simulink model "myo_sfun_one_myo_imu_emg"  (R2019a)
(part 6 of 12)

  "IW{2,1}(425,:)'" : Constant  Value=[1.908802925279713402773040797910653054714202880859375;-1.2138358984813477636777179213822819292545318603515625;0.01503844005797187570461215244677077862434089183807373046875;-1.5358594813991690575250004258123226463794708251953125;-0.59196391028480765950092745697475038468837738037109375;1.2715516743513524122732860632822848856449127197265625;1.2233297305976738034161144241807051002979278564453125;-0.5289314826547693026981278308085165917873382568359375]
      mask Display: e = 0.06;c1 = [120 150 230]/255;c2 = ([120 150 230]+0)/383;c3 = ([120 150 230]+128)/383;patch([0 1 1 0],[0 0 1 1],c1);patch([0 1 1 1-e 1-e 0+e],[0 0 1 1-e 0+e 0+e],c2);patch([0 0 1 1-e 0+e 0+e],[0 1 1 1-e 1-e 0+e],c3);plot([0 1 1 0 0],[0 0 1 1 0]);disp('weights');
  "IW{2,1}(426,:)'" : Constant  Value=[1.076656286956270580645877998904325067996978759765625;-0.8088007748125767282232345678494311869144439697265625;0.67060454814467396200683424467570148408412933349609375;0.88562860336622473145240519443177618086338043212890625;-1.9562657272639487615606412873603403568267822265625;-1.9554189585665968653671598076471127569675445556640625;-0.58641998996341160310663553900667466223239898681640625;0.269580957964742629062726564370677806437015533447265625]
      mask Display: e = 0.06;c1 = [120 150 230]/255;c2 = ([120 150 230]+0)/383;c3 = ([120 150 230]+128)/383;patch([0 1 1 0],[0 0 1 1],c1);patch([0 1 1 1-e 1-e 0+e],[0 0 1 1-e 0+e 0+e],c2);patch([0 0 1 1-e 0+e 0+e],[0 1 1 1-e 1-e 0+e],c3);plot([0 1 1 0 0],[0 0 1 1 0]);disp('weights');
  "IW{2,1}(427,:)'" : Constant  Value=[-0.721042740842791740618622498004697263240814208984375;0.79648621538253194795942135897348634898662567138671875;-0.53684047654335553811932868484291248023509979248046875;0.42689430211453827102019431549706496298313140869140625;2.549203011698739640422672891872934997081756591796875;0.3353743207324175745753791488823480904102325439453125;1.3664100055677750322757901813019998371601104736328125;-0.9924099379392383735165594771387986838817596435546875]
      mask Display: e = 0.06;c1 = [120 150 230]/255;c2 = ([120 150 230]+0)/383;c3 = ([120 150 230]+128)/383;patch([0 1 1 0],[0 0 1 1],c1);patch([0 1 1 1-e 1-e 0+e],[0 0 1 1-e 0+e 0+e],c2);patch([0 0 1 1-e 0+e 0+e],[0 1 1 1-e 1-e 0+e],c3);plot([0 1 1 0 0],[0 0 1 1 0]);disp('weights');
  "IW{2,1}(428,:)'" : Constant  Value=[1.2634311689343726836654013823135755956172943115234375;1.499519406449823843985313942539505660533905029296875;-0.8822519927699061792480961230467073619365692138671875;-0.0549891942636861752458088403727742843329906463623046875;-1.5362747666262255297198180414852686226367950439453125;-1.092163209413707480877064881497062742710113525390625;0.5684544617956106549172545783221721649169921875;1.6019203633066683156727094683446921408176422119140625]
      mask Display: e = 0.06;c1 = [120 150 230]/255;c2 = ([120 150 230]+0)/383;c3 = ([120 150 230]+128)/383;patch([0 1 1 0],[0 0 1 1],c1);patch([0 1 1 1-e 1-e 0+e],[0 0 1 1-e 0+e 0+e],c2);patch([0 0 1 1-e 0+e 0+e],[0 1 1 1-e 1-e 0+e],c3);plot([0 1 1 0 0],[0 0 1 1 0]);disp('weights');
  "IW{2,1}(429,:)'" : Constant  Value=[0.08693070549592145368489326529015670530498027801513671875;-1.518156541460599751047766403644345700740814208984375;-1.4111017266934429148506069395807571709156036376953125;2.2271029883890012257552371011115610599517822265625;-0.9991528979578829794405692155123688280582427978515625;0.024328099958265798907763866054665413685142993927001953125;-0.2054258345516097872263117096736095845699310302734375;0.7659566339452936745146871544420719146728515625]
      mask Display: e = 0.06;c1 = [120 150 230]/255;c2 = ([120 150 230]+0)/383;c3 = ([120 150 230]+128)/383;patch([0 1 1 0],[0 0 1 1],c1);patch([0 1 1 1-e 1-e 0+e],[0 0 1 1-e 0+e 0+e],c2);patch([0 0 1 1-e 0+e 0+e],[0 1 1 1-e 1-e 0+e],c3);plot([0 1 1 0 0],[0 0 1 1 0]);disp('weights');
  "IW{2,1}(43,:)'" : Constant  Value=[1.970097053050870794521642892505042254924774169921875;0.61319693162176391876272418812732212245464324951171875;-1.11470914765594297790585187613032758235931396484375;0.2366872070900522817549216370025533251464366912841796875;-1.507392518889222099431890455889515578746795654296875;1.7794743719183812036277458901167847216129302978515625;0.29415914149666377852554433047771453857421875;-0.66480034795872899877622330677695572376251220703125]
      mask Display: e = 0.06;c1 = [120 150 230]/255;c2 = ([120 150 230]+0)/383;c3 = ([120 150 230]+128)/383;patch([0 1 1 0],[0 0 1 1],c1);patch([0 1 1 1-e 1-e 0+e],[0 0 1 1-e 0+e 0+e],c2);patch([0 0 1 1-e 0+e 0+e],[0 1 1 1-e 1-e 0+e],c3);plot([0 1 1 0 0],[0 0 1 1 0]);disp('weights');
  "IW{2,1}(430,:)'" : Constant  Value=[0.91229328205142434793373240609071217477321624755859375;1.8134784160849555245675901460344903171062469482421875;1.8692781171544383678195799802779220044612884521484375;0.035866898596928382947357505372565356083214282989501953125;1.17660347229219208742279079160653054714202880859375;0.1717013531981310403562446253999951295554637908935546875;1.34724376949878621445577664417214691638946533203125;0.43452940443224041811021152170724235475063323974609375]
      mask Display: e = 0.06;c1 = [120 150 230]/255;c2 = ([120 150 230]+0)/383;c3 = ([120 150 230]+128)/383;patch([0 1 1 0],[0 0 1 1],c1);patch([0 1 1 1-e 1-e 0+e],[0 0 1 1-e 0+e 0+e],c2);patch([0 0 1 1-e 0+e 0+e],[0 1 1 1-e 1-e 0+e],c3);plot([0 1 1 0 0],[0 0 1 1 0]);disp('weights');
  "IW{2,1}(431,:)'" : Constant  Value=[1.7686581181827201181278041985933668911457061767578125;-1.601690710654345206620519093121401965618133544921875;-1.4180860902058913808332363259978592395782470703125;-1.18832699803570296381849402678199112415313720703125;0.2237601474155433700641282257493003271520137786865234375;0.65218668674513879945919825331657193601131439208984375;-0.88845803596487160636030466775991953909397125244140625;0.90809653286696201401895223170868121087551116943359375]
      mask Display: e = 0.06;c1 = [120 150 230]/255;c2 = ([120 150 230]+0)/383;c3 = ([120 150 230]+128)/383;patch([0 1 1 0],[0 0 1 1],c1);patch([0 1 1 1-e 1-e 0+e],[0 0 1 1-e 0+e 0+e],c2);patch([0 0 1 1-e 0+e 0+e],[0 1 1 1-e 1-e 0+e],c3);plot([0 1 1 0 0],[0 0 1 1 0]);disp('weights');
  "IW{2,1}(432,:)'" : Constant  Value=[-1.2080617079266013913496635723276995122432708740234375;0.72423144791304083778271660776226781308650970458984375;0.093387043987132101197090605637640692293643951416015625;0.2287847591571492145146038410530309192836284637451171875;1.0845655707055232852553672273643314838409423828125;2.143498846930034229529837830341421067714691162109375;1.7648296798747031832732545808539725840091705322265625;-0.01143002484406769637959033758534133085049688816070556640625]
      mask Display: e = 0.06;c1 = [120 150 230]/255;c2 = ([120 150 230]+0)/383;c3 = ([120 150 230]+128)/383;patch([0 1 1 0],[0 0 1 1],c1);patch([0 1 1 1-e 1-e 0+e],[0 0 1 1-e 0+e 0+e],c2);patch([0 0 1 1-e 0+e 0+e],[0 1 1 1-e 1-e 0+e],c3);plot([0 1 1 0 0],[0 0 1 1 0]);disp('weights');
  "IW{2,1}(433,:)'" : Constant  Value=[-0.5498636497147073587399290772737003862857818603515625;0.74773458564680994609119579763500951230525970458984375;0.350009369823531313326014924314222298562526702880859375;-0.503174198997705435232319359784014523029327392578125;1.3378549784211026807412281414144672453403472900390625;-0.56562537745451335613466881113708950579166412353515625;-1.7623422887645820988922196193016134202480316162109375;2.137193883301401253760332110687159001827239990234375]
      mask Display: e = 0.06;c1 = [120 150 230]/255;c2 = ([120 150 230]+0)/383;c3 = ([120 150 230]+128)/383;patch([0 1 1 0],[0 0 1 1],c1);patch([0 1 1 1-e 1-e 0+e],[0 0 1 1-e 0+e 0+e],c2);patch([0 0 1 1-e 0+e 0+e],[0 1 1 1-e 1-e 0+e],c3);plot([0 1 1 0 0],[0 0 1 1 0]);disp('weights');
  "IW{2,1}(434,:)'" : Constant  Value=[-1.684478970386725560359764131135307252407073974609375;1.6749987168562927575266030544298700988292694091796875;-1.2811478322068488022722476671333424746990203857421875;0.39101946305882961940625364150037057697772979736328125;0.476597130353781095468690409688861109316349029541015625;-0.038289527535806409941354644388411543332040309906005859375;-0.471648767075106445378906983023625798523426055908203125;1.755156876587362635433464674861170351505279541015625]
      mask Display: e = 0.06;c1 = [120 150 230]/255;c2 = ([120 150 230]+0)/383;c3 = ([120 150 230]+128)/383;patch([0 1 1 0],[0 0 1 1],c1);patch([0 1 1 1-e 1-e 0+e],[0 0 1 1-e 0+e 0+e],c2);patch([0 0 1 1-e 0+e 0+e],[0 1 1 1-e 1-e 0+e],c3);plot([0 1 1 0 0],[0 0 1 1 0]);disp('weights');
  "IW{2,1}(435,:)'" : Constant  Value=[-1.09749883271943016183058716706000268459320068359375;-0.7228536308750348471363622593344189226627349853515625;-0.91664807565766859287492707153433002531528472900390625;-0.1737902426546797107764774636962101794779300689697265625;1.86554391073935743605716197635047137737274169921875;1.67493352091046165952548108180053532123565673828125;0.328256548056097108290174446665332652628421783447265625;-1.47462782197953412577362541924230754375457763671875]
      mask Display: e = 0.06;c1 = [120 150 230]/255;c2 = ([120 150 230]+0)/383;c3 = ([120 150 230]+128)/383;patch([0 1 1 0],[0 0 1 1],c1);patch([0 1 1 1-e 1-e 0+e],[0 0 1 1-e 0+e 0+e],c2);patch([0 0 1 1-e 0+e 0+e],[0 1 1 1-e 1-e 0+e],c3);plot([0 1 1 0 0],[0 0 1 1 0]);disp('weights');
  "IW{2,1}(436,:)'" : Constant  Value=[-1.8622991051004882390174088868661783635616302490234375;1.5282596856373757976399474500794894993305206298828125;0.06699542167475343312776914217465673573315143585205078125;-0.89125276869858216510777992880321107804775238037109375;1.0063592161953760495407550479285418987274169921875;-1.647907139431842526988702957169152796268463134765625;-0.419451369693213449441060447497875429689884185791015625;-0.61184927408370726187314403432537801563739776611328125]
      mask Display: e = 0.06;c1 = [120 150 230]/255;c2 = ([120 150 230]+0)/383;c3 = ([120 150 230]+128)/383;patch([0 1 1 0],[0 0 1 1],c1);patch([0 1 1 1-e 1-e 0+e],[0 0 1 1-e 0+e 0+e],c2);patch([0 0 1 1-e 0+e 0+e],[0 1 1 1-e 1-e 0+e],c3);plot([0 1 1 0 0],[0 0 1 1 0]);disp('weights');
  "IW{2,1}(437,:)'" : Constant  Value=[-0.386335038572755029573357887784368358552455902099609375;0.67987513025270140953892905599786899983882904052734375;0.83342463915678799413200295020942576229572296142578125;-0.78544465833293397594161433517001569271087646484375;1.96444295468723684194856105023063719272613525390625;-1.2034402970973026025802710137213580310344696044921875;-1.084779028159589930879747043945826590061187744140625;1.5889814669219550768985982358572073280811309814453125]
      mask Display: e = 0.06;c1 = [120 150 230]/255;c2 = ([120 150 230]+0)/383;c3 = ([120 150 230]+128)/383;patch([0 1 1 0],[0 0 1 1],c1);patch([0 1 1 1-e 1-e 0+e],[0 0 1 1-e 0+e 0+e],c2);patch([0 0 1 1-e 0+e 0+e],[0 1 1 1-e 1-e 0+e],c3);plot([0 1 1 0 0],[0 0 1 1 0]);disp('weights');
  "IW{2,1}(438,:)'" : Constant  Value=[1.447670011134016387899237088277004659175872802734375;2.0249239545347190727397901355288922786712646484375;-1.3051959041181417919830209939391352236270904541015625;-0.272544054670654400940321693269652314484119415283203125;-0.270473658975852127017702741795801557600498199462890625;-1.0445512042442242073292391069117002189159393310546875;1.3405564141928929533520431505166925489902496337890625;0.244210291853415861762499616816057823598384857177734375]
      mask Display: e = 0.06;c1 = [120 150 230]/255;c2 = ([120 150 230]+0)/383;c3 = ([120 150 230]+128)/383;patch([0 1 1 0],[0 0 1 1],c1);patch([0 1 1 1-e 1-e 0+e],[0 0 1 1-e 0+e 0+e],c2);patch([0 0 1 1-e 0+e 0+e],[0 1 1 1-e 1-e 0+e],c3);plot([0 1 1 0 0],[0 0 1 1 0]);disp('weights');
  "IW{2,1}(439,:)'" : Constant  Value=[1.1959119026796216633812264262815006077289581298828125;0.47466445642241195113086860146722756326198577880859375;-0.723950913126099493410947616212069988250732421875;0.97731747065234486626650323159992694854736328125;-1.8300681987640621262158902027294971048831939697265625;0.471062294724000463208568589834612794220447540283203125;0.300068858348611910979997219328652136027812957763671875;2.00929184663641624553065412328578531742095947265625]
      mask Display: e = 0.06;c1 = [120 150 230]/255;c2 = ([120 150 230]+0)/383;c3 = ([120 150 230]+128)/383;patch([0 1 1 0],[0 0 1 1],c1);patch([0 1 1 1-e 1-e 0+e],[0 0 1 1-e 0+e 0+e],c2);patch([0 0 1 1-e 0+e 0+e],[0 1 1 1-e 1-e 0+e],c3);plot([0 1 1 0 0],[0 0 1 1 0]);disp('weights');
  "IW{2,1}(44,:)'" : Constant  Value=[1.5781069878844464771106004263856448233127593994140625;-1.7602350749520165873462929084780625998973846435546875;0.06590315742318096636775948127251467667520046234130859375;-1.45742290736087198865789105184376239776611328125;1.3106796571475543000673269489197991788387298583984375;0.31931782887147697191920769910211674869060516357421875;1.14325091964035951974665294983424246311187744140625;0.271731322341121239727357306037447415292263031005859375]
      mask Display: e = 0.06;c1 = [120 150 230]/255;c2 = ([120 150 230]+0)/383;c3 = ([120 150 230]+128)/383;patch([0 1 1 0],[0 0 1 1],c1);patch([0 1 1 1-e 1-e 0+e],[0 0 1 1-e 0+e 0+e],c2);patch([0 0 1 1-e 0+e 0+e],[0 1 1 1-e 1-e 0+e],c3);plot([0 1 1 0 0],[0 0 1 1 0]);disp('weights');
  "IW{2,1}(440,:)'" : Constant  Value=[0.2444979656170932214021007666815421544015407562255859375;0.25320953503716958632452360689057968556880950927734375;-0.91482335226723143772886714941705577075481414794921875;-1.1887452050953390969567635693238116800785064697265625;0.92946468491162048675136020392528735101222991943359375;-0.8795893241384338256949604328838177025318145751953125;-1.742588577134819960434697350137867033481597900390625;2.027252688550935655342755126184783875942230224609375]
      mask Display: e = 0.06;c1 = [120 150 230]/255;c2 = ([120 150 230]+0)/383;c3 = ([120 150 230]+128)/383;patch([0 1 1 0],[0 0 1 1],c1);patch([0 1 1 1-e 1-e 0+e],[0 0 1 1-e 0+e 0+e],c2);patch([0 0 1 1-e 0+e 0+e],[0 1 1 1-e 1-e 0+e],c3);plot([0 1 1 0 0],[0 0 1 1 0]);disp('weights');
  "IW{2,1}(441,:)'" : Constant  Value=[1.49083725976187952966256489162333309650421142578125;-0.1078297751313503083370193280643434263765811920166015625;-1.562790364440648005484035820700228214263916015625;-1.386522343669882584293873151182197034358978271484375;-0.9324292587433784529338254287722520530223846435546875;-0.62968018943971737488851658781641162931919097900390625;-1.7208674152053136108264652648358605802059173583984375;0.480021309574620913540599076441139914095401763916015625]
      mask Display: e = 0.06;c1 = [120 150 230]/255;c2 = ([120 150 230]+0)/383;c3 = ([120 150 230]+128)/383;patch([0 1 1 0],[0 0 1 1],c1);patch([0 1 1 1-e 1-e 0+e],[0 0 1 1-e 0+e 0+e],c2);patch([0 0 1 1-e 0+e 0+e],[0 1 1 1-e 1-e 0+e],c3);plot([0 1 1 0 0],[0 0 1 1 0]);disp('weights');
  "IW{2,1}(442,:)'" : Constant  Value=[1.419427784271670933691211757832206785678863525390625;-0.86184176357937769541450734323007054626941680908203125;-1.3930025465572726250940149839152581989765167236328125;1.502929121702403225668831510120071470737457275390625;0.1884602255780440105414896834190585650503635406494140625;-1.341648647949224670838930251193232834339141845703125;0.6584932340653060212076752577559091150760650634765625;1.5172526970433797277593157559749670326709747314453125]
      mask Display: e = 0.06;c1 = [120 150 230]/255;c2 = ([120 150 230]+0)/383;c3 = ([120 150 230]+128)/383;patch([0 1 1 0],[0 0 1 1],c1);patch([0 1 1 1-e 1-e 0+e],[0 0 1 1-e 0+e 0+e],c2);patch([0 0 1 1-e 0+e 0+e],[0 1 1 1-e 1-e 0+e],c3);plot([0 1 1 0 0],[0 0 1 1 0]);disp('weights');
  "IW{2,1}(443,:)'" : Constant  Value=[1.6942322735206591932666242428240366280078887939453125;0.68848747619682348908298763490165583789348602294921875;-0.6363648475862475617503832836518995463848114013671875;0.59618769558136530672953767862054519355297088623046875;-0.7665087115098796477496989609790034592151641845703125;1.0389542158220006484725672635249793529510498046875;1.971765654453049965155742029310204088687896728515625;1.1645173641494455107903149837511591613292694091796875]
      mask Display: e = 0.06;c1 = [120 150 230]/255;c2 = ([120 150 230]+0)/383;c3 = ([120 150 230]+128)/383;patch([0 1 1 0],[0 0 1 1],c1);patch([0 1 1 1-e 1-e 0+e],[0 0 1 1-e 0+e 0+e],c2);patch([0 0 1 1-e 0+e 0+e],[0 1 1 1-e 1-e 0+e],c3);plot([0 1 1 0 0],[0 0 1 1 0]);disp('weights');
  "IW{2,1}(444,:)'" : Constant  Value=[-1.1994870879449823775075856246985495090484619140625;-0.3536379564181846291148758609779179096221923828125;1.1820360403363654455688447342254221439361572265625;1.51940815251619998349497109302319586277008056640625;1.7996611921360383679058259076555259525775909423828125;-1.094775099300140386304747153189964592456817626953125;-0.0983590817533700756403192144716740585863590240478515625;1.1271969417472449404016288099228404462337493896484375]
      mask Display: e = 0.06;c1 = [120 150 230]/255;c2 = ([120 150 230]+0)/383;c3 = ([120 150 230]+128)/383;patch([0 1 1 0],[0 0 1 1],c1);patch([0 1 1 1-e 1-e 0+e],[0 0 1 1-e 0+e 0+e],c2);patch([0 0 1 1-e 0+e 0+e],[0 1 1 1-e 1-e 0+e],c3);plot([0 1 1 0 0],[0 0 1 1 0]);disp('weights');
  "IW{2,1}(445,:)'" : Constant  Value=[1.6460193434246515042929104311042465269565582275390625;0.95275031364290596602728555808425880968570709228515625;-0.8081658812080230180896478486829437315464019775390625;1.2554625798990202145688499513198621571063995361328125;0.88395409578853556542554770203423686325550079345703125;-0.81471698742909703927495002062642015516757965087890625;0.8740937417499849981794568520854227244853973388671875;1.7472164991341505579924842095351777970790863037109375]
      mask Display: e = 0.06;c1 = [120 150 230]/255;c2 = ([120 150 230]+0)/383;c3 = ([120 150 230]+128)/383;patch([0 1 1 0],[0 0 1 1],c1);patch([0 1 1 1-e 1-e 0+e],[0 0 1 1-e 0+e 0+e],c2);patch([0 0 1 1-e 0+e 0+e],[0 1 1 1-e 1-e 0+e],c3);plot([0 1 1 0 0],[0 0 1 1 0]);disp('weights');
  "IW{2,1}(446,:)'" : Constant  Value=[-0.418719574744047029479787624950404278934001922607421875;0.45752099612240748616187602237914688885211944580078125;0.7331671586043506660956836640252731740474700927734375;-1.6655488812604257731209145276807248592376708984375;-1.192074240287109176961166667751967906951904296875;1.25577071981947607781648912350647151470184326171875;-1.8239503457766357286118363845162093639373779296875;0.83910134010384418434824738142197020351886749267578125]
      mask Display: e = 0.06;c1 = [120 150 230]/255;c2 = ([120 150 230]+0)/383;c3 = ([120 150 230]+128)/383;patch([0 1 1 0],[0 0 1 1],c1);patch([0 1 1 1-e 1-e 0+e],[0 0 1 1-e 0+e 0+e],c2);patch([0 0 1 1-e 0+e 0+e],[0 1 1 1-e 1-e 0+e],c3);plot([0 1 1 0 0],[0 0 1 1 0]);disp('weights');
  "IW{2,1}(447,:)'" : Constant  Value=[1.6456347735626681849652186429011635482311248779296875;-1.7038432081545680230050265890895389020442962646484375;-0.433763112771412162604889317663037218153476715087890625;-0.30438289329319034859366865930496715009212493896484375;-0.95922777124080960131635720244958065450191497802734375;1.51918413581158429082051952718757092952728271484375;-0.99099576852023962825199987491942010819911956787109375;0.8451300769317244832024016432114876806735992431640625]
      mask Display: e = 0.06;c1 = [120 150 230]/255;c2 = ([120 150 230]+0)/383;c3 = ([120 150 230]+128)/383;patch([0 1 1 0],[0 0 1 1],c1);patch([0 1 1 1-e 1-e 0+e],[0 0 1 1-e 0+e 0+e],c2);patch([0 0 1 1-e 0+e 0+e],[0 1 1 1-e 1-e 0+e],c3);plot([0 1 1 0 0],[0 0 1 1 0]);disp('weights');
  "IW{2,1}(448,:)'" : Constant  Value=[1.3235678961511678775053724166355095803737640380859375;-0.2403985369923550552417879089261987246572971343994140625;0.37560522493124259835184375333483330905437469482421875;1.218658116879954178557454724796116352081298828125;1.6711138050380178743381520689581520855426788330078125;1.6525704067710662581447422780911438167095184326171875;1.3125992519337039698967828371678479015827178955078125;-0.5730686764621697459887172954040579497814178466796875]
      mask Display: e = 0.06;c1 = [120 150 230]/255;c2 = ([120 150 230]+0)/383;c3 = ([120 150 230]+128)/383;patch([0 1 1 0],[0 0 1 1],c1);patch([0 1 1 1-e 1-e 0+e],[0 0 1 1-e 0+e 0+e],c2);patch([0 0 1 1-e 0+e 0+e],[0 1 1 1-e 1-e 0+e],c3);plot([0 1 1 0 0],[0 0 1 1 0]);disp('weights');
  "IW{2,1}(449,:)'" : Constant  Value=[-0.27192590053676146677474889656878076493740081787109375;-1.245110113288279141130487914779223501682281494140625;0.10250989081913207401353105296948342584073543548583984375;-1.50718671441477436445666171493940055370330810546875;1.08693831376826022250270398217253386974334716796875;-1.84099998689164490173197918920777738094329833984375;0.7491758585288206262475796393118798732757568359375;-1.43360961212599935521438965224660933017730712890625]
      mask Display: e = 0.06;c1 = [120 150 230]/255;c2 = ([120 150 230]+0)/383;c3 = ([120 150 230]+128)/383;patch([0 1 1 0],[0 0 1 1],c1);patch([0 1 1 1-e 1-e 0+e],[0 0 1 1-e 0+e 0+e],c2);patch([0 0 1 1-e 0+e 0+e],[0 1 1 1-e 1-e 0+e],c3);plot([0 1 1 0 0],[0 0 1 1 0]);disp('weights');
  "IW{2,1}(45,:)'" : Constant  Value=[-2.058068747525070296688909365911968052387237548828125;-1.6974438370537330289522515158751048147678375244140625;0.67756823641316021866742858037468977272510528564453125;-0.54386372534373494946891014478751458227634429931640625;0.63814536885821093736836928655975498259067535400390625;-1.321737137397317241038763313554227352142333984375;-0.8913818029603373105373975704424083232879638671875;-0.4374724525263966601329457262181676924228668212890625]
      mask Display: e = 0.06;c1 = [120 150 230]/255;c2 = ([120 150 230]+0)/383;c3 = ([120 150 230]+128)/383;patch([0 1 1 0],[0 0 1 1],c1);patch([0 1 1 1-e 1-e 0+e],[0 0 1 1-e 0+e 0+e],c2);patch([0 0 1 1-e 0+e 0+e],[0 1 1 1-e 1-e 0+e],c3);plot([0 1 1 0 0],[0 0 1 1 0]);disp('weights');
  "IW{2,1}(450,:)'" : Constant  Value=[0.111819648022334738879379756326670758426189422607421875;0.68886207443856262155890135545632801949977874755859375;-1.81438059494320302889036611304618418216705322265625;-1.7745866170090824898153414324042387306690216064453125;0.493434270121383911078538631045375950634479522705078125;0.5891387028093599820266490496578626334667205810546875;1.820168318534121087992616594419814646244049072265625;0.5063195140962630791392484752577729523181915283203125]
      mask Display: e = 0.06;c1 = [120 150 230]/255;c2 = ([120 150 230]+0)/383;c3 = ([120 150 230]+128)/383;patch([0 1 1 0],[0 0 1 1],c1);patch([0 1 1 1-e 1-e 0+e],[0 0 1 1-e 0+e 0+e],c2);patch([0 0 1 1-e 0+e 0+e],[0 1 1 1-e 1-e 0+e],c3);plot([0 1 1 0 0],[0 0 1 1 0]);disp('weights');
  "IW{2,1}(451,:)'" : Constant  Value=[-1.5512918530885639878391657475731335580348968505859375;-1.416108168827626467844993385369889438152313232421875;0.88788180227700064239826360790175385773181915283203125;-0.1278119691545269720478472663671709597110748291015625;1.109324928308093927142863321932964026927947998046875;1.785026679497873747237690622569061815738677978515625;1.082422313592719120833862689323723316192626953125;0.344154249759374419870283645650488324463367462158203125]
      mask Display: e = 0.06;c1 = [120 150 230]/255;c2 = ([120 150 230]+0)/383;c3 = ([120 150 230]+128)/383;patch([0 1 1 0],[0 0 1 1],c1);patch([0 1 1 1-e 1-e 0+e],[0 0 1 1-e 0+e 0+e],c2);patch([0 0 1 1-e 0+e 0+e],[0 1 1 1-e 1-e 0+e],c3);plot([0 1 1 0 0],[0 0 1 1 0]);disp('weights');
  "IW{2,1}(452,:)'" : Constant  Value=[0.10900415859935246032375033564676414243876934051513671875;-1.7310874154853583828383989384747110307216644287109375;1.405467870878463809702907383325509727001190185546875;0.499111209860408966410005859870580025017261505126953125;0.55606589759542435214001443455344997346401214599609375;-1.59725125217449015480042362469248473644256591796875;1.632155344678247299583517815335653722286224365234375;-0.5408611905154139254392475777422077953815460205078125]
      mask Display: e = 0.06;c1 = [120 150 230]/255;c2 = ([120 150 230]+0)/383;c3 = ([120 150 230]+128)/383;patch([0 1 1 0],[0 0 1 1],c1);patch([0 1 1 1-e 1-e 0+e],[0 0 1 1-e 0+e 0+e],c2);patch([0 0 1 1-e 0+e 0+e],[0 1 1 1-e 1-e 0+e],c3);plot([0 1 1 0 0],[0 0 1 1 0]);disp('weights');
  "IW{2,1}(453,:)'" : Constant  Value=[1.346625396707150201791591825895011425018310546875;0.83847547019905011023155338989454321563243865966796875;1.90492255506132313058742511202581226825714111328125;1.2125613040568292699816765889408998191356658935546875;1.318708284019283194510308021563105285167694091796875;-0.27208910822183385302963642971008084714412689208984375;1.2289422596009191845922714492189697921276092529296875;0.178127453738075425260234396773739717900753021240234375]
      mask Display: e = 0.06;c1 = [120 150 230]/255;c2 = ([120 150 230]+0)/383;c3 = ([120 150 230]+128)/383;patch([0 1 1 0],[0 0 1 1],c1);patch([0 1 1 1-e 1-e 0+e],[0 0 1 1-e 0+e 0+e],c2);patch([0 0 1 1-e 0+e 0+e],[0 1 1 1-e 1-e 0+e],c3);plot([0 1 1 0 0],[0 0 1 1 0]);disp('weights');
  "IW{2,1}(454,:)'" : Constant  Value=[1.3636540746175338512102825916372239589691162109375;0.50817188833644466594563482431112788617610931396484375;-1.030658300962536078060338695649988949298858642578125;1.1732665168888003481839632513583637773990631103515625;-1.4554396962463929110498384034144692122936248779296875;0.21822274613665293419018098575179465115070343017578125;-1.9207801566961617556472674550605006515979766845703125;0.73016282423448763960749374746228568255901336669921875]
      mask Display: e = 0.06;c1 = [120 150 230]/255;c2 = ([120 150 230]+0)/383;c3 = ([120 150 230]+128)/383;patch([0 1 1 0],[0 0 1 1],c1);patch([0 1 1 1-e 1-e 0+e],[0 0 1 1-e 0+e 0+e],c2);patch([0 0 1 1-e 0+e 0+e],[0 1 1 1-e 1-e 0+e],c3);plot([0 1 1 0 0],[0 0 1 1 0]);disp('weights');
  "IW{2,1}(455,:)'" : Constant  Value=[-0.18999190046288105815364133377443067729473114013671875;0.57804807479159048266836862239870242774486541748046875;1.1855886884818176429945424388279207050800323486328125;-0.64094857152472695105416278238408267498016357421875;1.4244210827733516655513312798575498163700103759765625;-1.155547528042645932799814545433036983013153076171875;-1.626750741364674457400951723684556782245635986328125;1.6670500713903286804651315833325497806072235107421875]
      mask Display: e = 0.06;c1 = [120 150 230]/255;c2 = ([120 150 230]+0)/383;c3 = ([120 150 230]+128)/383;patch([0 1 1 0],[0 0 1 1],c1);patch([0 1 1 1-e 1-e 0+e],[0 0 1 1-e 0+e 0+e],c2);patch([0 0 1 1-e 0+e 0+e],[0 1 1 1-e 1-e 0+e],c3);plot([0 1 1 0 0],[0 0 1 1 0]);disp('weights');
  "IW{2,1}(456,:)'" : Constant  Value=[0.51659342651985806771364195810747332870960235595703125;-1.7673764990798310758890465876902453601360321044921875;-1.2005790743880024873391221262863837182521820068359375;-0.09356175604828008418589746497673331759870052337646484375;-0.80835226590308939531581700066453777253627777099609375;-1.881813429996495035112502591800875961780548095703125;-0.6010945349170897511470457175164483487606048583984375;1.2570754807005724007495928162825293838977813720703125]
      mask Display: e = 0.06;c1 = [120 150 230]/255;c2 = ([120 150 230]+0)/383;c3 = ([120 150 230]+128)/383;patch([0 1 1 0],[0 0 1 1],c1);patch([0 1 1 1-e 1-e 0+e],[0 0 1 1-e 0+e 0+e],c2);patch([0 0 1 1-e 0+e 0+e],[0 1 1 1-e 1-e 0+e],c3);plot([0 1 1 0 0],[0 0 1 1 0]);disp('weights');
  "IW{2,1}(457,:)'" : Constant  Value=[1.2889181834160619022355831475579179823398590087890625;-0.06234942018787816009339763922980637289583683013916015625;0.125520656183849277365283114704652689397335052490234375;0.2278346199585028208911552383142407052218914031982421875;1.364880359360622907871629649889655411243438720703125;-1.7551816178896668674269676557742059230804443359375;-1.6279057204772657829749960001208819448947906494140625;1.3904232954401891664275581206311471760272979736328125]
      mask Display: e = 0.06;c1 = [120 150 230]/255;c2 = ([120 150 230]+0)/383;c3 = ([120 150 230]+128)/383;patch([0 1 1 0],[0 0 1 1],c1);patch([0 1 1 1-e 1-e 0+e],[0 0 1 1-e 0+e 0+e],c2);patch([0 0 1 1-e 0+e 0+e],[0 1 1 1-e 1-e 0+e],c3);plot([0 1 1 0 0],[0 0 1 1 0]);disp('weights');
  "IW{2,1}(458,:)'" : Constant  Value=[-1.4765711804285828190330676079611293971538543701171875;-0.8401269807610936002362223007366992533206939697265625;1.667904378040498070134844965650700032711029052734375;-0.8668876328252548280062228513997979462146759033203125;-0.96308065287538624499319439564715139567852020263671875;0.6464737802231812491271512044477276504039764404296875;-1.817390079333127683725024326122365891933441162109375;0.0717015773478264784035474121992592699825763702392578125]
      mask Display: e = 0.06;c1 = [120 150 230]/255;c2 = ([120 150 230]+0)/383;c3 = ([120 150 230]+128)/383;patch([0 1 1 0],[0 0 1 1],c1);patch([0 1 1 1-e 1-e 0+e],[0 0 1 1-e 0+e 0+e],c2);patch([0 0 1 1-e 0+e 0+e],[0 1 1 1-e 1-e 0+e],c3);plot([0 1 1 0 0],[0 0 1 1 0]);disp('weights');
  "IW{2,1}(459,:)'" : Constant  Value=[1.4619893551682576759986886827391572296619415283203125;-0.478382253037435256626253021750017069280147552490234375;1.09894877037862670476897619664669036865234375;0.98370059070109860943631474583526141941547393798828125;0.33853452129109806723050724031054414808750152587890625;-1.8634608770444047731729142469703219830989837646484375;-0.84953969060517209310745556649635545909404754638671875;-1.54874483607171242738331784494221210479736328125]
      mask Display: e = 0.06;c1 = [120 150 230]/255;c2 = ([120 150 230]+0)/383;c3 = ([120 150 230]+128)/383;patch([0 1 1 0],[0 0 1 1],c1);patch([0 1 1 1-e 1-e 0+e],[0 0 1 1-e 0+e 0+e],c2);patch([0 0 1 1-e 0+e 0+e],[0 1 1 1-e 1-e 0+e],c3);plot([0 1 1 0 0],[0 0 1 1 0]);disp('weights');
  "IW{2,1}(46,:)'" : Constant  Value=[-0.29197737817094748802304593482404015958309173583984375;-0.3888894715460946560625643542152829468250274658203125;-0.471727977981710344668186962735489942133426666259765625;0.428481568131994394743600196306942962110042572021484375;-2.16380400911675252473287400789558887481689453125;-0.5652078136656708551299743703566491603851318359375;-2.175134104511693866612631609314121305942535400390625;-0.83728701906425284651191986995399929583072662353515625]
      mask Display: e = 0.06;c1 = [120 150 230]/255;c2 = ([120 150 230]+0)/383;c3 = ([120 150 230]+128)/383;patch([0 1 1 0],[0 0 1 1],c1);patch([0 1 1 1-e 1-e 0+e],[0 0 1 1-e 0+e 0+e],c2);patch([0 0 1 1-e 0+e 0+e],[0 1 1 1-e 1-e 0+e],c3);plot([0 1 1 0 0],[0 0 1 1 0]);disp('weights');
  "IW{2,1}(460,:)'" : Constant  Value=[-1.7410832317812043879001748791779391467571258544921875;1.1296530831303048802993771460023708641529083251953125;-0.6836633819173394410739774684770964086055755615234375;-1.682799515236981680033068187185563147068023681640625;0.421229283591670611297530513184028677642345428466796875;0.38530363946984247380811439143144525587558746337890625;-1.1595450073700550586153212861972860991954803466796875;1.29800016310675569997101774788461625576019287109375]
      mask Display: e = 0.06;c1 = [120 150 230]/255;c2 = ([120 150 230]+0)/383;c3 = ([120 150 230]+128)/383;patch([0 1 1 0],[0 0 1 1],c1);patch([0 1 1 1-e 1-e 0+e],[0 0 1 1-e 0+e 0+e],c2);patch([0 0 1 1-e 0+e 0+e],[0 1 1 1-e 1-e 0+e],c3);plot([0 1 1 0 0],[0 0 1 1 0]);disp('weights');
  "IW{2,1}(461,:)'" : Constant  Value=[-1.8263010335840601516821379846078343689441680908203125;-1.2286804200280021515112593988305889070034027099609375;0.65149677649490478348326405466650612652301788330078125;0.0505446179446576160376736197576974518597126007080078125;1.0271639902619018602791811645147390663623809814453125;1.694767574229393058971027130610309541225433349609375;-0.465269747824549717574171836531604640185832977294921875;-1.3817629626773364481806538606178946793079376220703125]
      mask Display: e = 0.06;c1 = [120 150 230]/255;c2 = ([120 150 230]+0)/383;c3 = ([120 150 230]+128)/383;patch([0 1 1 0],[0 0 1 1],c1);patch([0 1 1 1-e 1-e 0+e],[0 0 1 1-e 0+e 0+e],c2);patch([0 0 1 1-e 0+e 0+e],[0 1 1 1-e 1-e 0+e],c3);plot([0 1 1 0 0],[0 0 1 1 0]);disp('weights');
  "IW{2,1}(462,:)'" : Constant  Value=[1.60109400923383038417568968725390732288360595703125;-0.52522626644415104646412828515167348086833953857421875;-0.8661056410528742421917058891267515718936920166015625;1.023940112514241551622262704768218100070953369140625;-1.670246608526074982847831051913090050220489501953125;0.6527042656372332718461848344304598867893218994140625;-1.7618223640313555033998227372649125754833221435546875;-0.5463160315510233733249378929031081497669219970703125]
      mask Display: e = 0.06;c1 = [120 150 230]/255;c2 = ([120 150 230]+0)/383;c3 = ([120 150 230]+128)/383;patch([0 1 1 0],[0 0 1 1],c1);patch([0 1 1 1-e 1-e 0+e],[0 0 1 1-e 0+e 0+e],c2);patch([0 0 1 1-e 0+e 0+e],[0 1 1 1-e 1-e 0+e],c3);plot([0 1 1 0 0],[0 0 1 1 0]);disp('weights');
  "IW{2,1}(463,:)'" : Constant  Value=[-0.342830223214071694304294624089379794895648956298828125;-1.1867053959581961297686802936368621885776519775390625;1.70352758989853736437680709059350192546844482421875;-0.336017536470393396452749357194988988339900970458984375;1.89564020805277078096651166561059653759002685546875;-1.0914362614367065784648502813070081174373626708984375;-0.0360414198043656763825737243678304366767406463623046875;1.338994774159726564022321326774545013904571533203125]
      mask Display: e = 0.06;c1 = [120 150 230]/255;c2 = ([120 150 230]+0)/383;c3 = ([120 150 230]+128)/383;patch([0 1 1 0],[0 0 1 1],c1);patch([0 1 1 1-e 1-e 0+e],[0 0 1 1-e 0+e 0+e],c2);patch([0 0 1 1-e 0+e 0+e],[0 1 1 1-e 1-e 0+e],c3);plot([0 1 1 0 0],[0 0 1 1 0]);disp('weights');
  "IW{2,1}(464,:)'" : Constant  Value=[-1.84320234719937214862284236005507409572601318359375;0.89316531430534507052243498037569224834442138671875;1.278934109160143606231940793804824352264404296875;-1.3043551251196341400628853079979307949542999267578125;-1.35259215177986202860438424977473914623260498046875;-1.196791764988618833598366109072230756282806396484375;-0.481186031374078115874226568848825991153717041015625;0.16728291134412465179792661729152314364910125732421875]
      mask Display: e = 0.06;c1 = [120 150 230]/255;c2 = ([120 150 230]+0)/383;c3 = ([120 150 230]+128)/383;patch([0 1 1 0],[0 0 1 1],c1);patch([0 1 1 1-e 1-e 0+e],[0 0 1 1-e 0+e 0+e],c2);patch([0 0 1 1-e 0+e 0+e],[0 1 1 1-e 1-e 0+e],c3);plot([0 1 1 0 0],[0 0 1 1 0]);disp('weights');
  "IW{2,1}(465,:)'" : Constant  Value=[-0.495919288573932803831922910831053741276264190673828125;1.1288859466688914157117551440023817121982574462890625;0.59227314383006979259249646929674781858921051025390625;-0.434723589454314163216253064092597924172878265380859375;-1.1061240289423566185433855935116298496723175048828125;1.7251864346157261831393725515226833522319793701171875;-1.54622998393787458581982718897052109241485595703125;1.5975689431913255855732813870417885482311248779296875]
      mask Display: e = 0.06;c1 = [120 150 230]/255;c2 = ([120 150 230]+0)/383;c3 = ([120 150 230]+128)/383;patch([0 1 1 0],[0 0 1 1],c1);patch([0 1 1 1-e 1-e 0+e],[0 0 1 1-e 0+e 0+e],c2);patch([0 0 1 1-e 0+e 0+e],[0 1 1 1-e 1-e 0+e],c3);plot([0 1 1 0 0],[0 0 1 1 0]);disp('weights');
  "IW{2,1}(466,:)'" : Constant  Value=[-0.072622201688090692872634690502309240400791168212890625;1.8340735606872617946550008127815090119838714599609375;-0.6434647134475179885981788174831308424472808837890625;0.01331362047237333486038313168364766170270740985870361328125;0.67222917339024890193144301520078442990779876708984375;-0.5309847350764222984054185872082598507404327392578125;0.73061984761635156981895988792530260980129241943359375;2.44488847099693629161265562288463115692138671875]
      mask Display: e = 0.06;c1 = [120 150 230]/255;c2 = ([120 150 230]+0)/383;c3 = ([120 150 230]+128)/383;patch([0 1 1 0],[0 0 1 1],c1);patch([0 1 1 1-e 1-e 0+e],[0 0 1 1-e 0+e 0+e],c2);patch([0 0 1 1-e 0+e 0+e],[0 1 1 1-e 1-e 0+e],c3);plot([0 1 1 0 0],[0 0 1 1 0]);disp('weights');
  "IW{2,1}(467,:)'" : Constant  Value=[-0.6928974237817884240797638994990848004817962646484375;-1.6740146096956838306368808844126760959625244140625;-0.68028435490947181119025799489463679492473602294921875;0.06193748013113974104637549089602543972432613372802734375;-1.3950917275391161442854581764549948275089263916015625;-1.7880731985585918142334094227408058941364288330078125;-1.120528292446311358077082331874407827854156494140625;0.88233009208858559357935291700414381921291351318359375]
      mask Display: e = 0.06;c1 = [120 150 230]/255;c2 = ([120 150 230]+0)/383;c3 = ([120 150 230]+128)/383;patch([0 1 1 0],[0 0 1 1],c1);patch([0 1 1 1-e 1-e 0+e],[0 0 1 1-e 0+e 0+e],c2);patch([0 0 1 1-e 0+e 0+e],[0 1 1 1-e 1-e 0+e],c3);plot([0 1 1 0 0],[0 0 1 1 0]);disp('weights');
  "IW{2,1}(468,:)'" : Constant  Value=[-1.704651245745588017399541058694012463092803955078125;-0.205173281809027940880696405656635761260986328125;1.1352530457371210470540745518519543111324310302734375;-0.76237597125703959743958648687112145125865936279296875;-1.0187208403171312820489902151166461408138275146484375;-1.6648364167173654859510634196340106427669525146484375;-1.33262018868931164661262300796806812286376953125;-0.84380737968777885793514315082575194537639617919921875]
      mask Display: e = 0.06;c1 = [120 150 230]/255;c2 = ([120 150 230]+0)/383;c3 = ([120 150 230]+128)/383;patch([0 1 1 0],[0 0 1 1],c1);patch([0 1 1 1-e 1-e 0+e],[0 0 1 1-e 0+e 0+e],c2);patch([0 0 1 1-e 0+e 0+e],[0 1 1 1-e 1-e 0+e],c3);plot([0 1 1 0 0],[0 0 1 1 0]);disp('weights');
  "IW{2,1}(469,:)'" : Constant  Value=[1.0908746864454348379780412869877181947231292724609375;1.83760458957109573674415514688007533550262451171875;1.74516162696532450837594296899624168872833251953125;0.74928216227086574807714214330189861357212066650390625;0.92588665663726377186293348131584934890270233154296875;-0.63589564103393925176277434729854576289653778076171875;0.084056732324462257732733405646285973489284515380859375;1.2631646815478065892790482394048012793064117431640625]
      mask Display: e = 0.06;c1 = [120 150 230]/255;c2 = ([120 150 230]+0)/383;c3 = ([120 150 230]+128)/383;patch([0 1 1 0],[0 0 1 1],c1);patch([0 1 1 1-e 1-e 0+e],[0 0 1 1-e 0+e 0+e],c2);patch([0 0 1 1-e 0+e 0+e],[0 1 1 1-e 1-e 0+e],c3);plot([0 1 1 0 0],[0 0 1 1 0]);disp('weights');
  "IW{2,1}(47,:)'" : Constant  Value=[0.65759187738003033185663070980808697640895843505859375;1.1531124334303328726747395194252021610736846923828125;1.5337128087607820869919805772951804101467132568359375;-0.59958999157561343462674585680360905826091766357421875;-1.6007872022319791227573659853078424930572509765625;-0.443714726677683468647472864176961593329906463623046875;-1.948239914321326704538250851328484714031219482421875;0.06654690967011854529911119016105658374726772308349609375]
      mask Display: e = 0.06;c1 = [120 150 230]/255;c2 = ([120 150 230]+0)/383;c3 = ([120 150 230]+128)/383;patch([0 1 1 0],[0 0 1 1],c1);patch([0 1 1 1-e 1-e 0+e],[0 0 1 1-e 0+e 0+e],c2);patch([0 0 1 1-e 0+e 0+e],[0 1 1 1-e 1-e 0+e],c3);plot([0 1 1 0 0],[0 0 1 1 0]);disp('weights');
  "IW{2,1}(470,:)'" : Constant  Value=[-0.6307187321205649510602597729302942752838134765625;-0.45521010355887592258028462310903705656528472900390625;1.2121042430813140367007463282789103686809539794921875;-1.7406682388906362657365889390348456799983978271484375;-0.3726141659505000092167392722330987453460693359375;-1.624071883772505220377979640034027397632598876953125;-0.93727861109589849508694214819115586578845977783203125;1.462017083126777361457016013446263968944549560546875]
      mask Display: e = 0.06;c1 = [120 150 230]/255;c2 = ([120 150 230]+0)/383;c3 = ([120 150 230]+128)/383;patch([0 1 1 0],[0 0 1 1],c1);patch([0 1 1 1-e 1-e 0+e],[0 0 1 1-e 0+e 0+e],c2);patch([0 0 1 1-e 0+e 0+e],[0 1 1 1-e 1-e 0+e],c3);plot([0 1 1 0 0],[0 0 1 1 0]);disp('weights');
  "IW{2,1}(471,:)'" : Constant  Value=[2.05949162844077449108226574026048183441162109375;0.8462885695207120750893636795808561146259307861328125;1.975482353605422236597632945631630718708038330078125;-0.1855576478009340057884202224158798344433307647705078125;-0.5803752346740245204870234374538995325565338134765625;-0.8386081213190073047059058808372355997562408447265625;1.04999400780845153491327437222935259342193603515625;0.1710903874811346148110402509701089002192020416259765625]
      mask Display: e = 0.06;c1 = [120 150 230]/255;c2 = ([120 150 230]+0)/383;c3 = ([120 150 230]+128)/383;patch([0 1 1 0],[0 0 1 1],c1);patch([0 1 1 1-e 1-e 0+e],[0 0 1 1-e 0+e 0+e],c2);patch([0 0 1 1-e 0+e 0+e],[0 1 1 1-e 1-e 0+e],c3);plot([0 1 1 0 0],[0 0 1 1 0]);disp('weights');
  "IW{2,1}(472,:)'" : Constant  Value=[1.196372821319595214362152546527795493602752685546875;0.8497415704756814402998088553431443870067596435546875;0.70517330556419299814052692454424686729907989501953125;1.1739767989708713713525867206044495105743408203125;0.2795112137014876818597031160607002675533294677734375;-1.431463507054890893499532467103563249111175537109375;-0.85974655440916125659356339383521117269992828369140625;2.03924164862666668085466881166212260723114013671875]
      mask Display: e = 0.06;c1 = [120 150 230]/255;c2 = ([120 150 230]+0)/383;c3 = ([120 150 230]+128)/383;patch([0 1 1 0],[0 0 1 1],c1);patch([0 1 1 1-e 1-e 0+e],[0 0 1 1-e 0+e 0+e],c2);patch([0 0 1 1-e 0+e 0+e],[0 1 1 1-e 1-e 0+e],c3);plot([0 1 1 0 0],[0 0 1 1 0]);disp('weights');
  "IW{2,1}(473,:)'" : Constant  Value=[-1.569914891729929262709219983662478625774383544921875;0.71248998767843152446488375062472186982631683349609375;1.766504993464609984954449828364886343479156494140625;-1.39273449221400991149266701540909707546234130859375;1.324618316292147657264877125271596014499664306640625;0.98056472670050209838876753565273247659206390380859375;0.0657526915828758606874515635354327969253063201904296875;0.412439186302560489849611258250661194324493408203125]
      mask Display: e = 0.06;c1 = [120 150 230]/255;c2 = ([120 150 230]+0)/383;c3 = ([120 150 230]+128)/383;patch([0 1 1 0],[0 0 1 1],c1);patch([0 1 1 1-e 1-e 0+e],[0 0 1 1-e 0+e 0+e],c2);patch([0 0 1 1-e 0+e 0+e],[0 1 1 1-e 1-e 0+e],c3);plot([0 1 1 0 0],[0 0 1 1 0]);disp('weights');
  "IW{2,1}(474,:)'" : Constant  Value=[-1.496602636651553464020025785430334508419036865234375;2.284742414328153170544055683421902358531951904296875;1.44890632269699448642086281324736773967742919921875;-0.68583123159180547911972780639189295470714569091796875;-0.411301236946141013373079431403311900794506072998046875;-0.1867366403640671468355805018290993757545948028564453125;-0.45287477954424293358215436455793678760528564453125;-1.044791416654679228059876550105400383472442626953125]
      mask Display: e = 0.06;c1 = [120 150 230]/255;c2 = ([120 150 230]+0)/383;c3 = ([120 150 230]+128)/383;patch([0 1 1 0],[0 0 1 1],c1);patch([0 1 1 1-e 1-e 0+e],[0 0 1 1-e 0+e 0+e],c2);patch([0 0 1 1-e 0+e 0+e],[0 1 1 1-e 1-e 0+e],c3);plot([0 1 1 0 0],[0 0 1 1 0]);disp('weights');
  "IW{2,1}(475,:)'" : Constant  Value=[-1.2288938486461977728225747341639362275600433349609375;-0.163702288420320918316264169334317557513713836669921875;1.68767462910841548051621430204249918460845947265625;0.18457960052716615440004943593521602451801300048828125;-1.6897061246655056265808525495231151580810546875;1.1687286728810175606696475369972176849842071533203125;1.464728246009319168052797976997680962085723876953125;-0.33386188765047652982076442640391178429126739501953125]
      mask Display: e = 0.06;c1 = [120 150 230]/255;c2 = ([120 150 230]+0)/383;c3 = ([120 150 230]+128)/383;patch([0 1 1 0],[0 0 1 1],c1);patch([0 1 1 1-e 1-e 0+e],[0 0 1 1-e 0+e 0+e],c2);patch([0 0 1 1-e 0+e 0+e],[0 1 1 1-e 1-e 0+e],c3);plot([0 1 1 0 0],[0 0 1 1 0]);disp('weights');
  "IW{2,1}(476,:)'" : Constant  Value=[1.8112101836266620846771502328920178115367889404296875;-1.6196406582595253009770885910256765782833099365234375;0.850759610506119035022720709093846380710601806640625;0.4619087432528787839913775314926169812679290771484375;0.92203212450802585209430617396719753742218017578125;0.80789291393417650422037468160851858556270599365234375;-0.373283621770079399038166911850566975772380828857421875;-1.6120230653712095403307102969847619533538818359375]
      mask Display: e = 0.06;c1 = [120 150 230]/255;c2 = ([120 150 230]+0)/383;c3 = ([120 150 230]+128)/383;patch([0 1 1 0],[0 0 1 1],c1);patch([0 1 1 1-e 1-e 0+e],[0 0 1 1-e 0+e 0+e],c2);patch([0 0 1 1-e 0+e 0+e],[0 1 1 1-e 1-e 0+e],c3);plot([0 1 1 0 0],[0 0 1 1 0]);disp('weights');
  "IW{2,1}(477,:)'" : Constant  Value=[-1.02760011872689371870137620135210454463958740234375;0.66657815863905056641414148543844930827617645263671875;-1.5064137683900804542957985177054069936275482177734375;1.4863899533742586100970584084279835224151611328125;0.76120681507463749948527720334823243319988250732421875;-1.3916023257647622823895972032914869487285614013671875;-1.485101207786274191136044464656151831150054931640625;0.50338566011934648969372574356384575366973876953125]
      mask Display: e = 0.06;c1 = [120 150 230]/255;c2 = ([120 150 230]+0)/383;c3 = ([120 150 230]+128)/383;patch([0 1 1 0],[0 0 1 1],c1);patch([0 1 1 1-e 1-e 0+e],[0 0 1 1-e 0+e 0+e],c2);patch([0 0 1 1-e 0+e 0+e],[0 1 1 1-e 1-e 0+e],c3);plot([0 1 1 0 0],[0 0 1 1 0]);disp('weights');
  "IW{2,1}(478,:)'" : Constant  Value=[-0.7188111138938084732075139982043765485286712646484375;0.268513579013295700104180241396534256637096405029296875;-0.73213259439466404909779839726979844272136688232421875;1.4346558061020140417696211443399079144001007080078125;0.628616430632078060369849481503479182720184326171875;1.08108165527240718262191876419819891452789306640625;2.01237512894135672780748791410587728023529052734375;-1.518568895885144431900926065281964838504791259765625]
      mask Display: e = 0.06;c1 = [120 150 230]/255;c2 = ([120 150 230]+0)/383;c3 = ([120 150 230]+128)/383;patch([0 1 1 0],[0 0 1 1],c1);patch([0 1 1 1-e 1-e 0+e],[0 0 1 1-e 0+e 0+e],c2);patch([0 0 1 1-e 0+e 0+e],[0 1 1 1-e 1-e 0+e],c3);plot([0 1 1 0 0],[0 0 1 1 0]);disp('weights');
  "IW{2,1}(479,:)'" : Constant  Value=[-1.1726337223091654049511589619214646518230438232421875;0.6218159040198969478296930901706218719482421875;1.190851729517391266455206277896650135517120361328125;-1.0651230835900002968941180370165966451168060302734375;-1.25081826746582880360847411793656647205352783203125;-1.8471519624570602591262513669789768755435943603515625;0.50762171382490028914702406837022863328456878662109375;1.2043139502837132415180576572311110794544219970703125]
      mask Display: e = 0.06;c1 = [120 150 230]/255;c2 = ([120 150 230]+0)/383;c3 = ([120 150 230]+128)/383;patch([0 1 1 0],[0 0 1 1],c1);patch([0 1 1 1-e 1-e 0+e],[0 0 1 1-e 0+e 0+e],c2);patch([0 0 1 1-e 0+e 0+e],[0 1 1 1-e 1-e 0+e],c3);plot([0 1 1 0 0],[0 0 1 1 0]);disp('weights');
  "IW{2,1}(48,:)'" : Constant  Value=[1.989339141737506366780507960356771945953369140625;0.3510254126080589731628833760623820126056671142578125;1.1118933117981233404947261078632436692714691162109375;-0.56385536170020811308489783186814747750759124755859375;-0.315194469885802519559803158699651248753070831298828125;-0.1224662254762351187853397505023167468607425689697265625;-2.246873393464870360958229866810142993927001953125;-0.420826838617161247402265189521131105720996856689453125]
      mask Display: e = 0.06;c1 = [120 150 230]/255;c2 = ([120 150 230]+0)/383;c3 = ([120 150 230]+128)/383;patch([0 1 1 0],[0 0 1 1],c1);patch([0 1 1 1-e 1-e 0+e],[0 0 1 1-e 0+e 0+e],c2);patch([0 0 1 1-e 0+e 0+e],[0 1 1 1-e 1-e 0+e],c3);plot([0 1 1 0 0],[0 0 1 1 0]);disp('weights');
  "IW{2,1}(480,:)'" : Constant  Value=[0.06760197551004996918688760842996998690068721771240234375;-1.0166304546623974314201177548966370522975921630859375;-0.6592865783966941339855338810593821108341217041015625;-1.110314559386461841228310731821693480014801025390625;2.018369965522964548654272221028804779052734375;-1.5764810981949655133149690300342626869678497314453125;-0.5293966578283442192542906923335976898670196533203125;-1.21363686087833944071689984411932528018951416015625]
      mask Display: e = 0.06;c1 = [120 150 230]/255;c2 = ([120 150 230]+0)/383;c3 = ([120 150 230]+128)/383;patch([0 1 1 0],[0 0 1 1],c1);patch([0 1 1 1-e 1-e 0+e],[0 0 1 1-e 0+e 0+e],c2);patch([0 0 1 1-e 0+e 0+e],[0 1 1 1-e 1-e 0+e],c3);plot([0 1 1 0 0],[0 0 1 1 0]);disp('weights');
  "IW{2,1}(481,:)'" : Constant  Value=[1.6098863913930709923505446568015031516551971435546875;1.82285782333578705305399125791154801845550537109375;-0.64559056207255804959999068159959279000759124755859375;-1.4433700491998739945387342231697402894496917724609375;-1.4794473579069526980589444065117277204990386962890625;-0.36081906047284462157875850607524625957012176513671875;-0.81039814352502792527133124167448841035366058349609375;-0.174612114486950520397812169903772883117198944091796875]
      mask Display: e = 0.06;c1 = [120 150 230]/255;c2 = ([120 150 230]+0)/383;c3 = ([120 150 230]+128)/383;patch([0 1 1 0],[0 0 1 1],c1);patch([0 1 1 1-e 1-e 0+e],[0 0 1 1-e 0+e 0+e],c2);patch([0 0 1 1-e 0+e 0+e],[0 1 1 1-e 1-e 0+e],c3);plot([0 1 1 0 0],[0 0 1 1 0]);disp('weights');
  "IW{2,1}(482,:)'" : Constant  Value=[0.308396158862532576705461906385608017444610595703125;-1.483350088120044318884538370184600353240966796875;-1.4944739374719919755563068974879570305347442626953125;-1.238343462604848621566588917630724608898162841796875;0.97137409645041838945900281032663770020008087158203125;-1.9699037309863756117778166299103759229183197021484375;0.398619337709872623154438997516990639269351959228515625;-0.1000027184877689823139235159032978117465972900390625]
      mask Display: e = 0.06;c1 = [120 150 230]/255;c2 = ([120 150 230]+0)/383;c3 = ([120 150 230]+128)/383;patch([0 1 1 0],[0 0 1 1],c1);patch([0 1 1 1-e 1-e 0+e],[0 0 1 1-e 0+e 0+e],c2);patch([0 0 1 1-e 0+e 0+e],[0 1 1 1-e 1-e 0+e],c3);plot([0 1 1 0 0],[0 0 1 1 0]);disp('weights');
  "IW{2,1}(483,:)'" : Constant  Value=[-1.6946071244697211710672490880824625492095947265625;1.221048974397467734576139264390803873538970947265625;0.66259429745738651629238802343024872243404388427734375;-1.623927183722793099462933241738937795162200927734375;-1.520555614458623860940633676364086568355560302734375;-0.5711721868148427194711302945506758987903594970703125;-0.8011205150378846173708780042943544685840606689453125;0.64877638293491468601814631256274878978729248046875]
      mask Display: e = 0.06;c1 = [120 150 230]/255;c2 = ([120 150 230]+0)/383;c3 = ([120 150 230]+128)/383;patch([0 1 1 0],[0 0 1 1],c1);patch([0 1 1 1-e 1-e 0+e],[0 0 1 1-e 0+e 0+e],c2);patch([0 0 1 1-e 0+e 0+e],[0 1 1 1-e 1-e 0+e],c3);plot([0 1 1 0 0],[0 0 1 1 0]);disp('weights');
  "IW{2,1}(484,:)'" : Constant  Value=[-1.157574594575736082191497189342044293880462646484375;-0.84784166564671903376648742778343148529529571533203125;2.092292905105904932128169093630276620388031005859375;1.0929803623802938350451086080283857882022857666015625;-0.2002646277649058337289034170680679380893707275390625;-1.6635845931455026658341012080200016498565673828125;0.148661533248467814249949014993035234510898590087890625;-0.75183342188653179416490957009955309331417083740234375]
      mask Display: e = 0.06;c1 = [120 150 230]/255;c2 = ([120 150 230]+0)/383;c3 = ([120 150 230]+128)/383;patch([0 1 1 0],[0 0 1 1],c1);patch([0 1 1 1-e 1-e 0+e],[0 0 1 1-e 0+e 0+e],c2);patch([0 0 1 1-e 0+e 0+e],[0 1 1 1-e 1-e 0+e],c3);plot([0 1 1 0 0],[0 0 1 1 0]);disp('weights');
  "IW{2,1}(485,:)'" : Constant  Value=[2.128914554837456396541028880164958536624908447265625;0.7218889499550116273240973896463401615619659423828125;-1.3595415836741950865729222641675733029842376708984375;-1.511676005931837263318584518856368958950042724609375;0.67782303213338168657031701513915322721004486083984375;0.78804324216892929211297769143129698932170867919921875;-0.368437872762066354059840023182914592325687408447265625;-0.7578547600006506623770974329090677201747894287109375]
      mask Display: e = 0.06;c1 = [120 150 230]/255;c2 = ([120 150 230]+0)/383;c3 = ([120 150 230]+128)/383;patch([0 1 1 0],[0 0 1 1],c1);patch([0 1 1 1-e 1-e 0+e],[0 0 1 1-e 0+e 0+e],c2);patch([0 0 1 1-e 0+e 0+e],[0 1 1 1-e 1-e 0+e],c3);plot([0 1 1 0 0],[0 0 1 1 0]);disp('weights');
  "IW{2,1}(486,:)'" : Constant  Value=[1.4502856155797234638527015704312361776828765869140625;-1.393620362971380810535038108355365693569183349609375;-1.4983602416301893267558398292749188840389251708984375;-1.257399456324594044787090751924552023410797119140625;-1.275644110418096222048234267276711761951446533203125;-0.7519991947350721517295824014581739902496337890625;0.452753140322254277183589010746800340712070465087890625;-0.86565192897674736460800204440602101385593414306640625]
      mask Display: e = 0.06;c1 = [120 150 230]/255;c2 = ([120 150 230]+0)/383;c3 = ([120 150 230]+128)/383;patch([0 1 1 0],[0 0 1 1],c1);patch([0 1 1 1-e 1-e 0+e],[0 0 1 1-e 0+e 0+e],c2);patch([0 0 1 1-e 0+e 0+e],[0 1 1 1-e 1-e 0+e],c3);plot([0 1 1 0 0],[0 0 1 1 0]);disp('weights');
  "IW{2,1}(487,:)'" : Constant  Value=[0.822634457075106073631332037621177732944488525390625;-1.358248037122729900971762617700733244419097900390625;-0.1737158918737413682009673721040599048137664794921875;0.62920085138594405993472946647671051323413848876953125;-1.4131102749033506160714068755623884499073028564453125;1.44298292253273441332339643849991261959075927734375;-0.70401157600239161471478155363001860678195953369140625;-1.83315245430670614723567268811166286468505859375]
      mask Display: e = 0.06;c1 = [120 150 230]/255;c2 = ([120 150 230]+0)/383;c3 = ([120 150 230]+128)/383;patch([0 1 1 0],[0 0 1 1],c1);patch([0 1 1 1-e 1-e 0+e],[0 0 1 1-e 0+e 0+e],c2);patch([0 0 1 1-e 0+e 0+e],[0 1 1 1-e 1-e 0+e],c3);plot([0 1 1 0 0],[0 0 1 1 0]);disp('weights');
  "IW{2,1}(488,:)'" : Constant  Value=[-0.1845167929047638877282366820509196259081363677978515625;0.41835588251140876092648568373988382518291473388671875;-0.38019848651982190990139542918768711388111114501953125;-2.33630457949918035609471189673058688640594482421875;-0.4832677322238330130943495532847009599208831787109375;1.4317272155174141090583361801691353321075439453125;1.736165312631481327798610436730086803436279296875;-0.2379750162180374883913458461393020115792751312255859375]
      mask Display: e = 0.06;c1 = [120 150 230]/255;c2 = ([120 150 230]+0)/383;c3 = ([120 150 230]+128)/383;patch([0 1 1 0],[0 0 1 1],c1);patch([0 1 1 1-e 1-e 0+e],[0 0 1 1-e 0+e 0+e],c2);patch([0 0 1 1-e 0+e 0+e],[0 1 1 1-e 1-e 0+e],c3);plot([0 1 1 0 0],[0 0 1 1 0]);disp('weights');
  "IW{2,1}(489,:)'" : Constant  Value=[-1.71315522187115032437532136100344359874725341796875;-1.3751249494102193438038739259354770183563232421875;-0.75163730779787030211736009732703678309917449951171875;1.5161326026762489416199741754098795354366302490234375;-0.01207371183681381181240777067387170973233878612518310546875;-1.47748617955194649908889914513565599918365478515625;-1.00760322135796531739515558001585304737091064453125;0.509448666123086812973497217171825468540191650390625]
      mask Display: e = 0.06;c1 = [120 150 230]/255;c2 = ([120 150 230]+0)/383;c3 = ([120 150 230]+128)/383;patch([0 1 1 0],[0 0 1 1],c1);patch([0 1 1 1-e 1-e 0+e],[0 0 1 1-e 0+e 0+e],c2);patch([0 0 1 1-e 0+e 0+e],[0 1 1 1-e 1-e 0+e],c3);plot([0 1 1 0 0],[0 0 1 1 0]);disp('weights');
  "IW{2,1}(49,:)'" : Constant  Value=[-0.73084703892177571571409089301596395671367645263671875;1.6012928530430798890193955230643041431903839111328125;-0.080404434015713677208481158231734298169612884521484375;-0.453680866110419966918954060020041652023792266845703125;1.2697789724477781536648990368121303617954254150390625;-1.6935366528426227805681492100120522081851959228515625;1.337834163059698600051206085481680929660797119140625;-1.21244109021384804947274460573680698871612548828125]
      mask Display: e = 0.06;c1 = [120 150 230]/255;c2 = ([120 150 230]+0)/383;c3 = ([120 150 230]+128)/383;patch([0 1 1 0],[0 0 1 1],c1);patch([0 1 1 1-e 1-e 0+e],[0 0 1 1-e 0+e 0+e],c2);patch([0 0 1 1-e 0+e 0+e],[0 1 1 1-e 1-e 0+e],c3);plot([0 1 1 0 0],[0 0 1 1 0]);disp('weights');
  "IW{2,1}(490,:)'" : Constant  Value=[1.861198028271384696807899672421626746654510498046875;1.72717971125945712884686145116575062274932861328125;-0.1370697129883551024231991277702036313712596893310546875;-0.826173810754017523549919133074581623077392578125;-1.2657469080503627179012937631341628730297088623046875;-0.44224382591335398284826396775315515697002410888671875;-1.1102012036082540280546027133823372423648834228515625;1.097199491751585487264719631639309227466583251953125]
      mask Display: e = 0.06;c1 = [120 150 230]/255;c2 = ([120 150 230]+0)/383;c3 = ([120 150 230]+128)/383;patch([0 1 1 0],[0 0 1 1],c1);patch([0 1 1 1-e 1-e 0+e],[0 0 1 1-e 0+e 0+e],c2);patch([0 0 1 1-e 0+e 0+e],[0 1 1 1-e 1-e 0+e],c3);plot([0 1 1 0 0],[0 0 1 1 0]);disp('weights');
  "IW{2,1}(491,:)'" : Constant  Value=[-0.75955597882400471831942923017777502536773681640625;0.71408219339101208777975671182502992451190948486328125;-1.6967825555472828558123410402913577854633331298828125;0.7341110136379220829638825307483784854412078857421875;-0.5592312105818166845239147733082063496112823486328125;0.85986314990457268780943422825657762587070465087890625;-1.74733364422455306197434765635989606380462646484375;1.5721897216687421572345328968367539346218109130859375]
      mask Display: e = 0.06;c1 = [120 150 230]/255;c2 = ([120 150 230]+0)/383;c3 = ([120 150 230]+128)/383;patch([0 1 1 0],[0 0 1 1],c1);patch([0 1 1 1-e 1-e 0+e],[0 0 1 1-e 0+e 0+e],c2);patch([0 0 1 1-e 0+e 0+e],[0 1 1 1-e 1-e 0+e],c3);plot([0 1 1 0 0],[0 0 1 1 0]);disp('weights');
  "IW{2,1}(492,:)'" : Constant  Value=[1.54514795283253913993348760413937270641326904296875;0.08210181255613656359226837366804829798638820648193359375;1.03872009218692795684546581469476222991943359375;0.72341041747982071097311518315109424293041229248046875;1.399948078818173513582223677076399326324462890625;1.4861027383982021721209321185597218573093414306640625;0.8640333903548105265457479617907665669918060302734375;-1.44795804357926893857211325666867196559906005859375]
      mask Display: e = 0.06;c1 = [120 150 230]/255;c2 = ([120 150 230]+0)/383;c3 = ([120 150 230]+128)/383;patch([0 1 1 0],[0 0 1 1],c1);patch([0 1 1 1-e 1-e 0+e],[0 0 1 1-e 0+e 0+e],c2);patch([0 0 1 1-e 0+e 0+e],[0 1 1 1-e 1-e 0+e],c3);plot([0 1 1 0 0],[0 0 1 1 0]);disp('weights');
  "IW{2,1}(493,:)'" : Constant  Value=[-0.3245980381096063016599373440840281546115875244140625;0.163031781555113719495153645766549743711948394775390625;-0.414079476495472997843450002619647420942783355712890625;-0.2230892493828474931749639154077158309519290924072265625;0.08776818235214615959716155657588387839496135711669921875;1.530121008804143034609523965627886354923248291015625;1.7938176978261781702173038866021670401096343994140625;-2.225301941957096740765109643689356744289398193359375]
      mask Display: e = 0.06;c1 = [120 150 230]/255;c2 = ([120 150 230]+0)/383;c3 = ([120 150 230]+128)/383;patch([0 1 1 0],[0 0 1 1],c1);patch([0 1 1 1-e 1-e 0+e],[0 0 1 1-e 0+e 0+e],c2);patch([0 0 1 1-e 0+e 0+e],[0 1 1 1-e 1-e 0+e],c3);plot([0 1 1 0 0],[0 0 1 1 0]);disp('weights');
  "IW{2,1}(494,:)'" : Constant  Value=[-1.266405505087220273452430774341337382793426513671875;0.160393291429333284536795645180973224341869354248046875;0.242786468376962327742063507685088552534580230712890625;-0.53162450380059411703115301861544139683246612548828125;-1.7893300606367759097992120587150566279888153076171875;1.9059325853911832648890367636340670287609100341796875;-0.931559424177998973704006857587955892086029052734375;1.183127314034374766293922220938839018344879150390625]
      mask Display: e = 0.06;c1 = [120 150 230]/255;c2 = ([120 150 230]+0)/383;c3 = ([120 150 230]+128)/383;patch([0 1 1 0],[0 0 1 1],c1);patch([0 1 1 1-e 1-e 0+e],[0 0 1 1-e 0+e 0+e],c2);patch([0 0 1 1-e 0+e 0+e],[0 1 1 1-e 1-e 0+e],c3);plot([0 1 1 0 0],[0 0 1 1 0]);disp('weights');
  "IW{2,1}(495,:)'" : Constant  Value=[-0.70908826918114031823137111132382415235042572021484375;1.637437501880628420991570237674750387668609619140625;0.455498587605101812325614218934788368642330169677734375;-0.347552777441448357276243541491567157208919525146484375;1.7041781679066005938949501796741969883441925048828125;1.8470974404941780111499838312738575041294097900390625;0.7783528340278460522227987894439138472080230712890625;0.7986860540572136013537374310544691979885101318359375]
      mask Display: e = 0.06;c1 = [120 150 230]/255;c2 = ([120 150 230]+0)/383;c3 = ([120 150 230]+128)/383;patch([0 1 1 0],[0 0 1 1],c1);patch([0 1 1 1-e 1-e 0+e],[0 0 1 1-e 0+e 0+e],c2);patch([0 0 1 1-e 0+e 0+e],[0 1 1 1-e 1-e 0+e],c3);plot([0 1 1 0 0],[0 0 1 1 0]);disp('weights');
  "IW{2,1}(496,:)'" : Constant  Value=[-0.070014899899124516391424322137027047574520111083984375;1.66714078540710897158305670018307864665985107421875;0.9553410826642803055364083775202743709087371826171875;-1.16234904046259668319862612406723201274871826171875;1.6330031607986883468441874356358312070369720458984375;0.59200942324606342648252166327438317239284515380859375;1.6790341534228476749746050700196065008640289306640625;0.2416284540569455518976837993250228464603424072265625]
      mask Display: e = 0.06;c1 = [120 150 230]/255;c2 = ([120 150 230]+0)/383;c3 = ([120 150 230]+128)/383;patch([0 1 1 0],[0 0 1 1],c1);patch([0 1 1 1-e 1-e 0+e],[0 0 1 1-e 0+e 0+e],c2);patch([0 0 1 1-e 0+e 0+e],[0 1 1 1-e 1-e 0+e],c3);plot([0 1 1 0 0],[0 0 1 1 0]);disp('weights');
  "IW{2,1}(497,:)'" : Constant  Value=[1.32857077742367568617964934674091637134552001953125;1.7725982804872331133339002917637117207050323486328125;-0.62063637669645610461799378754221834242343902587890625;0.6693552122285553185321305136312730610370635986328125;-0.395125675851767776958212152749183587729930877685546875;1.3639490378048562124746467816294170916080474853515625;-1.6361253662742092362947232686565257608890533447265625;0.55492878246055943325387715958640910685062408447265625]
      mask Display: e = 0.06;c1 = [120 150 230]/255;c2 = ([120 150 230]+0)/383;c3 = ([120 150 230]+128)/383;patch([0 1 1 0],[0 0 1 1],c1);patch([0 1 1 1-e 1-e 0+e],[0 0 1 1-e 0+e 0+e],c2);patch([0 0 1 1-e 0+e 0+e],[0 1 1 1-e 1-e 0+e],c3);plot([0 1 1 0 0],[0 0 1 1 0]);disp('weights');
  "IW{2,1}(498,:)'" : Constant  Value=[1.8017436798640307227259427236276678740978240966796875;0.787954426121096229707063685054890811443328857421875;1.05599332112906996172796425526030361652374267578125;-0.82251893831696920589280352942296303808689117431640625;0.495643583555207045687751588047831319272518157958984375;-1.13579560460711359581864599022082984447479248046875;1.7521388723847757251661505506490357220172882080078125;-0.93513523592179759180709197607939131557941436767578125]
      mask Display: e = 0.06;c1 = [120 150 230]/255;c2 = ([120 150 230]+0)/383;c3 = ([120 150 230]+128)/383;patch([0 1 1 0],[0 0 1 1],c1);patch([0 1 1 1-e 1-e 0+e],[0 0 1 1-e 0+e 0+e],c2);patch([0 0 1 1-e 0+e 0+e],[0 1 1 1-e 1-e 0+e],c3);plot([0 1 1 0 0],[0 0 1 1 0]);disp('weights');
  "IW{2,1}(499,:)'" : Constant  Value=[-0.6237672624429138057422505880822427570819854736328125;0.27031293122476662826869642231031320989131927490234375;-0.4376813283034675094995691324584186077117919921875;0.57840103112499996473871988200698979198932647705078125;0.815267234021921805009469608194194734096527099609375;1.89808520589676010814628170919604599475860595703125;1.39773321769982228346407282515428960323333740234375;1.9419776780554105499732031603343784809112548828125]
      mask Display: e = 0.06;c1 = [120 150 230]/255;c2 = ([120 150 230]+0)/383;c3 = ([120 150 230]+128)/383;patch([0 1 1 0],[0 0 1 1],c1);patch([0 1 1 1-e 1-e 0+e],[0 0 1 1-e 0+e 0+e],c2);patch([0 0 1 1-e 0+e 0+e],[0 1 1 1-e 1-e 0+e],c3);plot([0 1 1 0 0],[0 0 1 1 0]);disp('weights');
  "IW{2,1}(5,:)'" : Constant  Value=[-0.16563936181678762249447345311637036502361297607421875;-0.007226205257817530647201920146471820771694183349609375;-1.599481669259194660526191000826656818389892578125;-1.9690186615978604312005018073250539600849151611328125;-1.5846939096168721761159758898429572582244873046875;0.0274247585518724579234373095459886826574802398681640625;0.5557498493434545050462247672840021550655364990234375;-1.3438275745683796458251890726387500762939453125]
      mask Display: e = 0.06;c1 = [120 150 230]/255;c2 = ([120 150 230]+0)/383;c3 = ([120 150 230]+128)/383;patch([0 1 1 0],[0 0 1 1],c1);patch([0 1 1 1-e 1-e 0+e],[0 0 1 1-e 0+e 0+e],c2);patch([0 0 1 1-e 0+e 0+e],[0 1 1 1-e 1-e 0+e],c3);plot([0 1 1 0 0],[0 0 1 1 0]);disp('weights');
  "IW{2,1}(50,:)'" : Constant  Value=[-0.76324824974984994963023154923575930297374725341796875;0.416049359064521062645525262269075028598308563232421875;-1.3547237892572103756805290686315856873989105224609375;-1.84324866077664495378485298715531826019287109375;-0.56035580948326291217398420485551469027996063232421875;0.430902038635862627558026360929943621158599853515625;-2.10192241402107971026680388604290783405303955078125;0.349355798602189182577859583034296520054340362548828125]
      mask Display: e = 0.06;c1 = [120 150 230]/255;c2 = ([120 150 230]+0)/383;c3 = ([120 150 230]+128)/383;patch([0 1 1 0],[0 0 1 1],c1);patch([0 1 1 1-e 1-e 0+e],[0 0 1 1-e 0+e 0+e],c2);patch([0 0 1 1-e 0+e 0+e],[0 1 1 1-e 1-e 0+e],c3);plot([0 1 1 0 0],[0 0 1 1 0]);disp('weights');
  "IW{2,1}(500,:)'" : Constant  Value=[-0.313104776347255919777268218240351416170597076416015625;0.57303508122144197756142602884210646152496337890625;0.6113964002496545813158945748000405728816986083984375;1.8782268986203611849106209774618037045001983642578125;1.156476240494380025580767323845066130161285400390625;-1.83946434016351378915032910299487411975860595703125;-0.541420782886920637366756636765785515308380126953125;-1.3103467923067746436771585649694316089153289794921875]
      mask Display: e = 0.06;c1 = [120 150 230]/255;c2 = ([120 150 230]+0)/383;c3 = ([120 150 230]+128)/383;patch([0 1 1 0],[0 0 1 1],c1);patch([0 1 1 1-e 1-e 0+e],[0 0 1 1-e 0+e 0+e],c2);patch([0 0 1 1-e 0+e 0+e],[0 1 1 1-e 1-e 0+e],c3);plot([0 1 1 0 0],[0 0 1 1 0]);disp('weights');
  "IW{2,1}(501,:)'" : Constant  Value=[1.4790491154180085420222212633234448730945587158203125;0.681491031065608598993321720627136528491973876953125;-0.26357926267902753725280717844725586473941802978515625;0.68261502577031019090014751782291568815708160400390625;-1.245288445143598377029547918937169015407562255859375;-1.10170214487960915761277647106908261775970458984375;-2.197253460508464595335453850566409528255462646484375;-0.18501159661989652338576206602738238871097564697265625]
      mask Display: e = 0.06;c1 = [120 150 230]/255;c2 = ([120 150 230]+0)/383;c3 = ([120 150 230]+128)/383;patch([0 1 1 0],[0 0 1 1],c1);patch([0 1 1 1-e 1-e 0+e],[0 0 1 1-e 0+e 0+e],c2);patch([0 0 1 1-e 0+e 0+e],[0 1 1 1-e 1-e 0+e],c3);plot([0 1 1 0 0],[0 0 1 1 0]);disp('weights');
  "IW{2,1}(502,:)'" : Constant  Value=[-0.51178815551607692579949571154429577291011810302734375;0.79696638035322353577072362895705737173557281494140625;0.5805513845755350121891069647972472012042999267578125;-1.2602401903004627481408306266530416905879974365234375;1.4571131629140741114980528436717577278614044189453125;-1.594938220777011306239501209347508847713470458984375;-0.273719038631936972816305342348641715943813323974609375;1.8960874135176479793329917811206541955471038818359375]
      mask Display: e = 0.06;c1 = [120 150 230]/255;c2 = ([120 150 230]+0)/383;c3 = ([120 150 230]+128)/383;patch([0 1 1 0],[0 0 1 1],c1);patch([0 1 1 1-e 1-e 0+e],[0 0 1 1-e 0+e 0+e],c2);patch([0 0 1 1-e 0+e 0+e],[0 1 1 1-e 1-e 0+e],c3);plot([0 1 1 0 0],[0 0 1 1 0]);disp('weights');
  "IW{2,1}(503,:)'" : Constant  Value=[1.1258109309791588525939687315258197486400604248046875;0.408170152926930374093217324116267263889312744140625;0.8426336717644480334143963773385621607303619384765625;0.5086324008109366356933378483518026769161224365234375;1.6544485469636700525342121181893162429332733154296875;1.437181967514224556481394756701774895191192626953125;1.7344801118434032272119793560705147683620452880859375;-0.8992909562915609722466570019605569541454315185546875]
      mask Display: e = 0.06;c1 = [120 150 230]/255;c2 = ([120 150 230]+0)/383;c3 = ([120 150 230]+128)/383;patch([0 1 1 0],[0 0 1 1],c1);patch([0 1 1 1-e 1-e 0+e],[0 0 1 1-e 0+e 0+e],c2);patch([0 0 1 1-e 0+e 0+e],[0 1 1 1-e 1-e 0+e],c3);plot([0 1 1 0 0],[0 0 1 1 0]);disp('weights');
  "IW{2,1}(504,:)'" : Constant  Value=[-1.986052519514175163095615062047727406024932861328125;-1.688627966051614581743933740654028952121734619140625;-0.06861616180594685976412705485927290283143520355224609375;0.36550869213349546082980623395997099578380584716796875;-0.0452393273778826376929629304868285544216632843017578125;-0.81149196158417424840081366710364818572998046875;1.335113754666826135775181683129630982875823974609375;-1.2217662104111541854223332848050631582736968994140625]
      mask Display: e = 0.06;c1 = [120 150 230]/255;c2 = ([120 150 230]+0)/383;c3 = ([120 150 230]+128)/383;patch([0 1 1 0],[0 0 1 1],c1);patch([0 1 1 1-e 1-e 0+e],[0 0 1 1-e 0+e 0+e],c2);patch([0 0 1 1-e 0+e 0+e],[0 1 1 1-e 1-e 0+e],c3);plot([0 1 1 0 0],[0 0 1 1 0]);disp('weights');
  "IW{2,1}(505,:)'" : Constant  Value=[-1.097870804326036786591203053831122815608978271484375;0.39428925361889588518948812634334899485111236572265625;0.58251500851229565114408615045249462127685546875;1.5598205735321284404193420414230786263942718505859375;-1.05516375408520701739689684472978115081787109375;-0.835890193635706157948561667581088840961456298828125;2.168373810497051135115498254890553653240203857421875;0.81645898488446266849649646246689371764659881591796875]
      mask Display: e = 0.06;c1 = [120 150 230]/255;c2 = ([120 150 230]+0)/383;c3 = ([120 150 230]+128)/383;patch([0 1 1 0],[0 0 1 1],c1);patch([0 1 1 1-e 1-e 0+e],[0 0 1 1-e 0+e 0+e],c2);patch([0 0 1 1-e 0+e 0+e],[0 1 1 1-e 1-e 0+e],c3);plot([0 1 1 0 0],[0 0 1 1 0]);disp('weights');
  "IW{2,1}(506,:)'" : Constant  Value=[1.9135499701385605408887613521073944866657257080078125;0.269418158591238576793358561189961619675159454345703125;-1.0263955571781628872685132591868750751018524169921875;-0.31326718956206123234409233191399835050106048583984375;-0.61957933934089048921833864369546063244342803955078125;-1.8357516462827321301887195659219287335872650146484375;-0.420716261996193108263497606458258815109729766845703125;1.4267869702564743850103923250571824610233306884765625]
      mask Display: e = 0.06;c1 = [120 150 230]/255;c2 = ([120 150 230]+0)/383;c3 = ([120 150 230]+128)/383;patch([0 1 1 0],[0 0 1 1],c1);patch([0 1 1 1-e 1-e 0+e],[0 0 1 1-e 0+e 0+e],c2);patch([0 0 1 1-e 0+e 0+e],[0 1 1 1-e 1-e 0+e],c3);plot([0 1 1 0 0],[0 0 1 1 0]);disp('weights');
  "IW{2,1}(507,:)'" : Constant  Value=[-0.150777507787159092966788875855854712426662445068359375;-1.84073331581798793621373988571576774120330810546875;-0.5881109631589132025197841358021833002567291259765625;-0.569217713806215552807543645030818879604339599609375;-1.1483453983252649432955649899668060243129730224609375;0.94439355334078900483518737019039690494537353515625;-1.8220343276557546818850141789880581200122833251953125;-1.1446427130091214596774307210580445826053619384765625]
      mask Display: e = 0.06;c1 = [120 150 230]/255;c2 = ([120 150 230]+0)/383;c3 = ([120 150 230]+128)/383;patch([0 1 1 0],[0 0 1 1],c1);patch([0 1 1 1-e 1-e 0+e],[0 0 1 1-e 0+e 0+e],c2);patch([0 0 1 1-e 0+e 0+e],[0 1 1 1-e 1-e 0+e],c3);plot([0 1 1 0 0],[0 0 1 1 0]);disp('weights');
  "IW{2,1}(508,:)'" : Constant  Value=[1.491790172469844577562980703078210353851318359375;-1.4930480750871979456206872782786376774311065673828125;0.2380837743141342166541818414771114476025104522705078125;-1.667028604672200042813301479327492415904998779296875;-0.79768861806650048773548178360215388238430023193359375;-0.357934450997786923753807286630035378038883209228515625;-1.0570937106378839320797169420984573662281036376953125;-1.3625655094291533320216558422544039785861968994140625]
      mask Display: e = 0.06;c1 = [120 150 230]/255;c2 = ([120 150 230]+0)/383;c3 = ([120 150 230]+128)/383;patch([0 1 1 0],[0 0 1 1],c1);patch([0 1 1 1-e 1-e 0+e],[0 0 1 1-e 0+e 0+e],c2);patch([0 0 1 1-e 0+e 0+e],[0 1 1 1-e 1-e 0+e],c3);plot([0 1 1 0 0],[0 0 1 1 0]);disp('weights');
  "IW{2,1}(509,:)'" : Constant  Value=[-0.76506440683042786776724142328021116554737091064453125;2.14839508744180829324932346935383975505828857421875;0.894577723096715349271335071534849703311920166015625;1.5224111549664318676633456561830826103687286376953125;-0.001979658152352328261136538145592567161656916141510009765625;1.1731753779631670653316177777014672756195068359375;0.6657825496695426448212629111367277801036834716796875;0.97669988223814174777004382121958769857883453369140625]
      mask Display: e = 0.06;c1 = [120 150 230]/255;c2 = ([120 150 230]+0)/383;c3 = ([120 150 230]+128)/383;patch([0 1 1 0],[0 0 1 1],c1);patch([0 1 1 1-e 1-e 0+e],[0 0 1 1-e 0+e 0+e],c2);patch([0 0 1 1-e 0+e 0+e],[0 1 1 1-e 1-e 0+e],c3);plot([0 1 1 0 0],[0 0 1 1 0]);disp('weights');
  "IW{2,1}(51,:)'" : Constant  Value=[-0.270416107588409115880523359010112471878528594970703125;0.115510163182885816635092623982927761971950531005859375;-0.4308574055634954991234053522930480539798736572265625;1.764696411276891918618048293865285813808441162109375;-1.91804347956707488265237770974636077880859375;-0.99892599314099606022665511773084290325641632080078125;-0.57822084520888783476522121418383903801441192626953125;1.7316421346029671202160216125776059925556182861328125]
      mask Display: e = 0.06;c1 = [120 150 230]/255;c2 = ([120 150 230]+0)/383;c3 = ([120 150 230]+128)/383;patch([0 1 1 0],[0 0 1 1],c1);patch([0 1 1 1-e 1-e 0+e],[0 0 1 1-e 0+e 0+e],c2);patch([0 0 1 1-e 0+e 0+e],[0 1 1 1-e 1-e 0+e],c3);plot([0 1 1 0 0],[0 0 1 1 0]);disp('weights');
  "IW{2,1}(510,:)'" : Constant  Value=[-1.1294311594423207534276798469363711774349212646484375;1.475621075257439684946803026832640171051025390625;0.6403583893418935968355754084768705070018768310546875;-0.69935643702778171881817570465500466525554656982421875;-1.539801398046500846561457365169189870357513427734375;-1.194589231718778510327183539629913866519927978515625;1.452312438318084986121903057210147380828857421875;-0.80591105007193741815996190780424512922763824462890625]
      mask Display: e = 0.06;c1 = [120 150 230]/255;c2 = ([120 150 230]+0)/383;c3 = ([120 150 230]+128)/383;patch([0 1 1 0],[0 0 1 1],c1);patch([0 1 1 1-e 1-e 0+e],[0 0 1 1-e 0+e 0+e],c2);patch([0 0 1 1-e 0+e 0+e],[0 1 1 1-e 1-e 0+e],c3);plot([0 1 1 0 0],[0 0 1 1 0]);disp('weights');
  "IW{2,1}(511,:)'" : Constant  Value=[0.73613827619807181701361287196050398051738739013671875;1.842774875696976177863461998640559613704681396484375;-0.87421548115440483872617960514617152512073516845703125;-1.69355266765983092369651785702444612979888916015625;-0.0120729515538387059681024737756160902790725231170654296875;0.55725944864203647011180464687640778720378875732421875;1.561432027464954241935402023955248296260833740234375;0.8403302009772632974460293553420342504978179931640625]
      mask Display: e = 0.06;c1 = [120 150 230]/255;c2 = ([120 150 230]+0)/383;c3 = ([120 150 230]+128)/383;patch([0 1 1 0],[0 0 1 1],c1);patch([0 1 1 1-e 1-e 0+e],[0 0 1 1-e 0+e 0+e],c2);patch([0 0 1 1-e 0+e 0+e],[0 1 1 1-e 1-e 0+e],c3);plot([0 1 1 0 0],[0 0 1 1 0]);disp('weights');
  "IW{2,1}(512,:)'" : Constant  Value=[1.0632914899570249378513153715175576508045196533203125;1.590625637458683794278613277128897607326507568359375;1.736303870567482920961310810525901615619659423828125;0.59339651386957081857786988621228374540805816650390625;0.80389352780436096335137108326307497918605804443359375;1.6322497276336973559551779544563032686710357666015625;0.63809414540475872801295054159709252417087554931640625;0.57889031143579738891702390901627950370311737060546875]
      mask Display: e = 0.06;c1 = [120 150 230]/255;c2 = ([120 150 230]+0)/383;c3 = ([120 150 230]+128)/383;patch([0 1 1 0],[0 0 1 1],c1);patch([0 1 1 1-e 1-e 0+e],[0 0 1 1-e 0+e 0+e],c2);patch([0 0 1 1-e 0+e 0+e],[0 1 1 1-e 1-e 0+e],c3);plot([0 1 1 0 0],[0 0 1 1 0]);disp('weights');
  "IW{2,1}(513,:)'" : Constant  Value=[-0.82421694745751483690554550776141695678234100341796875;0.30188432932277009523858168904553167521953582763671875;-1.567438925959779627561374582001008093357086181640625;-0.120190389102396155696084178998717106878757476806640625;-1.6389442003140983761255711215198971331119537353515625;0.8309751255576058870389033472747541964054107666015625;1.0917322147940742294025540104485116899013519287109375;1.7027661611578019940083095207228325307369232177734375]
      mask Display: e = 0.06;c1 = [120 150 230]/255;c2 = ([120 150 230]+0)/383;c3 = ([120 150 230]+128)/383;patch([0 1 1 0],[0 0 1 1],c1);patch([0 1 1 1-e 1-e 0+e],[0 0 1 1-e 0+e 0+e],c2);patch([0 0 1 1-e 0+e 0+e],[0 1 1 1-e 1-e 0+e],c3);plot([0 1 1 0 0],[0 0 1 1 0]);disp('weights');
  "IW{2,1}(514,:)'" : Constant  Value=[0.15790438026419717498782802067580632865428924560546875;-2.00753335625779971707061122287996113300323486328125;0.6640213078966024085048047709278762340545654296875;1.0916200405024889530380960422917269170284271240234375;-1.122105618555867767582867600140161812305450439453125;1.5386700693944093121245941802044399082660675048828125;0.2922821342582271331167476091650314629077911376953125;-1.2148700648903141274814743155729956924915313720703125]
      mask Display: e = 0.06;c1 = [120 150 230]/255;c2 = ([120 150 230]+0)/383;c3 = ([120 150 230]+128)/383;patch([0 1 1 0],[0 0 1 1],c1);patch([0 1 1 1-e 1-e 0+e],[0 0 1 1-e 0+e 0+e],c2);patch([0 0 1 1-e 0+e 0+e],[0 1 1 1-e 1-e 0+e],c3);plot([0 1 1 0 0],[0 0 1 1 0]);disp('weights');
  "IW{2,1}(515,:)'" : Constant  Value=[-1.554753130981170183844142229645512998104095458984375;1.9187829605312820557827535594697110354900360107421875;-0.5083128594857500015535833881585858762264251708984375;-0.1576099188749150725730174826821894384920597076416015625;-1.3569638600881350765092747678863815963268280029296875;1.261472734879882207081891465350054204463958740234375;-0.53956175932050276511375841437256895005702972412109375;1.081026487982526429476592966238968074321746826171875]
      mask Display: e = 0.06;c1 = [120 150 230]/255;c2 = ([120 150 230]+0)/383;c3 = ([120 150 230]+128)/383;patch([0 1 1 0],[0 0 1 1],c1);patch([0 1 1 1-e 1-e 0+e],[0 0 1 1-e 0+e 0+e],c2);patch([0 0 1 1-e 0+e 0+e],[0 1 1 1-e 1-e 0+e],c3);plot([0 1 1 0 0],[0 0 1 1 0]);disp('weights');
  "IW{2,1}(516,:)'" : Constant  Value=[-0.36487137537473801618403967950143851339817047119140625;-0.293203795033078196130560399979003705084323883056640625;0.68254800317010400068085118618910200893878936767578125;1.5039752748932488923827577309566549956798553466796875;1.41832001311092792406043372466228902339935302734375;1.6437776661162535329907541381544433534145355224609375;-1.2672352569096683172489292701357044279575347900390625;-1.30152076032857877407877822406589984893798828125]
      mask Display: e = 0.06;c1 = [120 150 230]/255;c2 = ([120 150 230]+0)/383;c3 = ([120 150 230]+128)/383;patch([0 1 1 0],[0 0 1 1],c1);patch([0 1 1 1-e 1-e 0+e],[0 0 1 1-e 0+e 0+e],c2);patch([0 0 1 1-e 0+e 0+e],[0 1 1 1-e 1-e 0+e],c3);plot([0 1 1 0 0],[0 0 1 1 0]);disp('weights');
  "IW{2,1}(517,:)'" : Constant  Value=[-1.1892425533219626032632731948979198932647705078125;-0.7548168819471172685808824098785407841205596923828125;1.480614388430722794254279506276361644268035888671875;-0.67148710365231512042782924254424870014190673828125;-1.38907897371924615725902185658924281597137451171875;-1.380778631834774561326639741309918463230133056640625;-1.120750573583021658663483322015963494777679443359375;-1.176522048471383197210116122732870280742645263671875]
      mask Display: e = 0.06;c1 = [120 150 230]/255;c2 = ([120 150 230]+0)/383;c3 = ([120 150 230]+128)/383;patch([0 1 1 0],[0 0 1 1],c1);patch([0 1 1 1-e 1-e 0+e],[0 0 1 1-e 0+e 0+e],c2);patch([0 0 1 1-e 0+e 0+e],[0 1 1 1-e 1-e 0+e],c3);plot([0 1 1 0 0],[0 0 1 1 0]);disp('weights');
  "IW{2,1}(518,:)'" : Constant  Value=[1.482715736409068174594949596212245523929595947265625;-1.342400526473154886986094425083138048648834228515625;-1.4134417557615870375542499459697864949703216552734375;0.6686741370533726414038255825289525091648101806640625;1.58651505404211956573590214247815310955047607421875;-0.6224791437195371646140529264812357723712921142578125;-0.69133329772313134586880778442719019949436187744140625;1.062792335344026728449762231321074068546295166015625]
      mask Display: e = 0.06;c1 = [120 150 230]/255;c2 = ([120 150 230]+0)/383;c3 = ([120 150 230]+128)/383;patch([0 1 1 0],[0 0 1 1],c1);patch([0 1 1 1-e 1-e 0+e],[0 0 1 1-e 0+e 0+e],c2);patch([0 0 1 1-e 0+e 0+e],[0 1 1 1-e 1-e 0+e],c3);plot([0 1 1 0 0],[0 0 1 1 0]);disp('weights');
  "IW{2,1}(519,:)'" : Constant  Value=[-0.388195802982468529673809598534717224538326263427734375;-1.88020972311264156218157950206659734249114990234375;-0.61695810454045652004850808225455693900585174560546875;0.79499476327360429905866112676449120044708251953125;1.8195035387977427365768789968569763004779815673828125;-0.60831214670204636352224270012811757624149322509765625;-1.5984957388229812380586736253462731838226318359375;-0.0587060619950559026136716056498698890209197998046875]
      mask Display: e = 0.06;c1 = [120 150 230]/255;c2 = ([120 150 230]+0)/383;c3 = ([120 150 230]+128)/383;patch([0 1 1 0],[0 0 1 1],c1);patch([0 1 1 1-e 1-e 0+e],[0 0 1 1-e 0+e 0+e],c2);patch([0 0 1 1-e 0+e 0+e],[0 1 1 1-e 1-e 0+e],c3);plot([0 1 1 0 0],[0 0 1 1 0]);disp('weights');
  "IW{2,1}(52,:)'" : Constant  Value=[1.536266886460530667335433463449589908123016357421875;-0.8854349973556134845154019785695709288120269775390625;-0.741564361520239412328692196751944720745086669921875;-0.89748392347244865252520185094908811151981353759765625;0.74024994845556724154533867476857267320156097412109375;-1.28208704251387306527476539486087858676910400390625;1.364436088226878229789917895686812698841094970703125;-1.5710055389724899566061822042684070765972137451171875]
      mask Display: e = 0.06;c1 = [120 150 230]/255;c2 = ([120 150 230]+0)/383;c3 = ([120 150 230]+128)/383;patch([0 1 1 0],[0 0 1 1],c1);patch([0 1 1 1-e 1-e 0+e],[0 0 1 1-e 0+e 0+e],c2);patch([0 0 1 1-e 0+e 0+e],[0 1 1 1-e 1-e 0+e],c3);plot([0 1 1 0 0],[0 0 1 1 0]);disp('weights');
  "IW{2,1}(520,:)'" : Constant  Value=[0.5348031248189848430030224335496313869953155517578125;1.1047582701849985031827827697270549833774566650390625;0.55386145720178581175474619158194400370121002197265625;1.080873722872972120256918060476891696453094482421875;1.767105047284687646680367834051139652729034423828125;1.3291148661940799247105360336718149483203887939453125;1.6282344253456451088624135081772692501544952392578125;0.70783874034256244467400165376602672040462493896484375]
      mask Display: e = 0.06;c1 = [120 150 230]/255;c2 = ([120 150 230]+0)/383;c3 = ([120 150 230]+128)/383;patch([0 1 1 0],[0 0 1 1],c1);patch([0 1 1 1-e 1-e 0+e],[0 0 1 1-e 0+e 0+e],c2);patch([0 0 1 1-e 0+e 0+e],[0 1 1 1-e 1-e 0+e],c3);plot([0 1 1 0 0],[0 0 1 1 0]);disp('weights');
  "IW{2,1}(521,:)'" : Constant  Value=[0.986078097980417123125107536907307803630828857421875;1.831813655619013214703727498999796807765960693359375;0.0837348964500722880988092811094247736036777496337890625;-0.374310859603177725762890304395114071667194366455078125;0.01469120969215030429733115369117513182573020458221435546875;2.331545618531454255872858993825502693653106689453125;-0.77256515785341495217153351404704153537750244140625;-0.85326336581069950337763430070481263101100921630859375]
      mask Display: e = 0.06;c1 = [120 150 230]/255;c2 = ([120 150 230]+0)/383;c3 = ([120 150 230]+128)/383;patch([0 1 1 0],[0 0 1 1],c1);patch([0 1 1 1-e 1-e 0+e],[0 0 1 1-e 0+e 0+e],c2);patch([0 0 1 1-e 0+e 0+e],[0 1 1 1-e 1-e 0+e],c3);plot([0 1 1 0 0],[0 0 1 1 0]);disp('weights');
  "IW{2,1}(522,:)'" : Constant  Value=[0.1066469450560699472330128401154070161283016204833984375;-0.5945334244902229503537682830938138067722320556640625;0.130231994653638605274892370289308018982410430908203125;1.652139337173611721709676203317940235137939453125;0.37148864978641282785787325337878428399562835693359375;0.99288216391501460389434896569582633674144744873046875;2.32339278013373107256711591617204248905181884765625;1.17675854499267718011878969264216721057891845703125]
      mask Display: e = 0.06;c1 = [120 150 230]/255;c2 = ([120 150 230]+0)/383;c3 = ([120 150 230]+128)/383;patch([0 1 1 0],[0 0 1 1],c1);patch([0 1 1 1-e 1-e 0+e],[0 0 1 1-e 0+e 0+e],c2);patch([0 0 1 1-e 0+e 0+e],[0 1 1 1-e 1-e 0+e],c3);plot([0 1 1 0 0],[0 0 1 1 0]);disp('weights');
  "IW{2,1}(523,:)'" : Constant  Value=[1.1947698025783581865510996067314408719539642333984375;0.207670754946080726721646669830079190433025360107421875;-0.60478968762722351559801836629048921167850494384765625;-0.328816096571413918336901360817137174308300018310546875;1.470846178773699275410535847186110913753509521484375;0.0638969454981070106303064903841004706919193267822265625;-2.17467869089696730355854015215300023555755615234375;-1.4858576375495140542426497631822712719440460205078125]
      mask Display: e = 0.06;c1 = [120 150 230]/255;c2 = ([120 150 230]+0)/383;c3 = ([120 150 230]+128)/383;patch([0 1 1 0],[0 0 1 1],c1);patch([0 1 1 1-e 1-e 0+e],[0 0 1 1-e 0+e 0+e],c2);patch([0 0 1 1-e 0+e 0+e],[0 1 1 1-e 1-e 0+e],c3);plot([0 1 1 0 0],[0 0 1 1 0]);disp('weights');
  "IW{2,1}(524,:)'" : Constant  Value=[-1.5189431230263525929302659278619103133678436279296875;1.1296727439074751853098632636829279363155364990234375;1.5123108446710957775138695069472305476665496826171875;0.2038844216481283944109037520320271141827106475830078125;0.433783273623665588392128711348050273954868316650390625;-2.154210404886420793246770699624903500080108642578125;-0.263790184648224623753520745594869367778301239013671875;0.58530229247478982035346461998415179550647735595703125]
      mask Display: e = 0.06;c1 = [120 150 230]/255;c2 = ([120 150 230]+0)/383;c3 = ([120 150 230]+128)/383;patch([0 1 1 0],[0 0 1 1],c1);patch([0 1 1 1-e 1-e 0+e],[0 0 1 1-e 0+e 0+e],c2);patch([0 0 1 1-e 0+e 0+e],[0 1 1 1-e 1-e 0+e],c3);plot([0 1 1 0 0],[0 0 1 1 0]);disp('weights');
  "IW{2,1}(525,:)'" : Constant  Value=[0.53917622471561532648820502799935638904571533203125;1.134444910461219091502016453887335956096649169921875;1.7252370857969889783589678700082004070281982421875;1.798917183799744190508818064699880778789520263671875;-0.0279686515112925505877061738146949210204184055328369140625;-0.80176049428341433777944757821387611329555511474609375;-1.2070593015911625922598204851965419948101043701171875;1.033460066081169248519699976895935833454132080078125]
      mask Display: e = 0.06;c1 = [120 150 230]/255;c2 = ([120 150 230]+0)/383;c3 = ([120 150 230]+128)/383;patch([0 1 1 0],[0 0 1 1],c1);patch([0 1 1 1-e 1-e 0+e],[0 0 1 1-e 0+e 0+e],c2);patch([0 0 1 1-e 0+e 0+e],[0 1 1 1-e 1-e 0+e],c3);plot([0 1 1 0 0],[0 0 1 1 0]);disp('weights');
  "IW{2,1}(526,:)'" : Constant  Value=[-0.71181713253930378737521778020891360938549041748046875;-1.716288187743292947828877004212699830532073974609375;-0.5814640512016067130929286577156744897365570068359375;1.3060622072168708296402428459259681403636932373046875;-1.1230631976390281767663736900431104004383087158203125;0.432498180483566085907654041875503025949001312255859375;1.105003114410923359400840126909315586090087890625;1.625622919553234790868145864806137979030609130859375]
      mask Display: e = 0.06;c1 = [120 150 230]/255;c2 = ([120 150 230]+0)/383;c3 = ([120 150 230]+128)/383;patch([0 1 1 0],[0 0 1 1],c1);patch([0 1 1 1-e 1-e 0+e],[0 0 1 1-e 0+e 0+e],c2);patch([0 0 1 1-e 0+e 0+e],[0 1 1 1-e 1-e 0+e],c3);plot([0 1 1 0 0],[0 0 1 1 0]);disp('weights');
  "IW{2,1}(527,:)'" : Constant  Value=[1.157635955111781189685871140682138502597808837890625;-0.38261973660885839620959814055822789669036865234375;-1.8663137244174838880184097433811984956264495849609375;-1.6644746771058358536521382120554335415363311767578125;-0.9383262778484624533348323893733322620391845703125;1.3469057022274617541057750713662244379520416259765625;-0.78489709588202061230077788422931917011737823486328125;0.03756997074073901987656398659964906983077526092529296875]
      mask Display: e = 0.06;c1 = [120 150 230]/255;c2 = ([120 150 230]+0)/383;c3 = ([120 150 230]+128)/383;patch([0 1 1 0],[0 0 1 1],c1);patch([0 1 1 1-e 1-e 0+e],[0 0 1 1-e 0+e 0+e],c2);patch([0 0 1 1-e 0+e 0+e],[0 1 1 1-e 1-e 0+e],c3);plot([0 1 1 0 0],[0 0 1 1 0]);disp('weights');
  "IW{2,1}(528,:)'" : Constant  Value=[1.08737074048125936798214752343483269214630126953125;-0.53387910810381600246188327218987978994846343994140625;0.7346159464670887206949601022643037140369415283203125;-0.439921745311730727490129311263444833457469940185546875;-2.051249004403752795866466840379871428012847900390625;0.06812066509880192188841618872174876742064952850341796875;-1.743801921416689548749445748399011790752410888671875;1.2495224054864007001697245868854224681854248046875]
      mask Display: e = 0.06;c1 = [120 150 230]/255;c2 = ([120 150 230]+0)/383;c3 = ([120 150 230]+128)/383;patch([0 1 1 0],[0 0 1 1],c1);patch([0 1 1 1-e 1-e 0+e],[0 0 1 1-e 0+e 0+e],c2);patch([0 0 1 1-e 0+e 0+e],[0 1 1 1-e 1-e 0+e],c3);plot([0 1 1 0 0],[0 0 1 1 0]);disp('weights');
  "IW{2,1}(529,:)'" : Constant  Value=[0.186015066512516258345755204572924412786960601806640625;1.695718484977229767451945008360780775547027587890625;-1.6830684995440459150728429449372924864292144775390625;-0.1513411817628505795507720677051111124455928802490234375;1.37304995253624095852273967466317117214202880859375;0.1290726342584104513466769503793329931795597076416015625;1.697247726071997586672068791813217103481292724609375;0.65890895497847157269433182591455988585948944091796875]
      mask Display: e = 0.06;c1 = [120 150 230]/255;c2 = ([120 150 230]+0)/383;c3 = ([120 150 230]+128)/383;patch([0 1 1 0],[0 0 1 1],c1);patch([0 1 1 1-e 1-e 0+e],[0 0 1 1-e 0+e 0+e],c2);patch([0 0 1 1-e 0+e 0+e],[0 1 1 1-e 1-e 0+e],c3);plot([0 1 1 0 0],[0 0 1 1 0]);disp('weights');
  "IW{2,1}(53,:)'" : Constant  Value=[1.1311120412194932693950022439821623265743255615234375;-0.03761833601437176988202537586403195746243000030517578125;-1.4205314511537492361270551555207930505275726318359375;-0.6786888632526710818382298384676687419414520263671875;-0.862185019523606488434097627759911119937896728515625;-2.249661705792425525629596450016833841800689697265625;0.8755720058851625964280174230225384235382080078125;-0.82926523464061163704030832377611659467220306396484375]
      mask Display: e = 0.06;c1 = [120 150 230]/255;c2 = ([120 150 230]+0)/383;c3 = ([120 150 230]+128)/383;patch([0 1 1 0],[0 0 1 1],c1);patch([0 1 1 1-e 1-e 0+e],[0 0 1 1-e 0+e 0+e],c2);patch([0 0 1 1-e 0+e 0+e],[0 1 1 1-e 1-e 0+e],c3);plot([0 1 1 0 0],[0 0 1 1 0]);disp('weights');
  "IW{2,1}(530,:)'" : Constant  Value=[1.0990168628454302091057570578414015471935272216796875;-1.917798228586485631552704944624565541744232177734375;-0.61349505909448354135093950390000827610492706298828125;0.46166766674287973426515918617951683700084686279296875;-0.890315700943348442564229117124341428279876708984375;1.81739222433423464053703355602920055389404296875;-0.00204481335883934488284463526497347629629075527191162109375;1.245106226810837046770075176027603447437286376953125]
      mask Display: e = 0.06;c1 = [120 150 230]/255;c2 = ([120 150 230]+0)/383;c3 = ([120 150 230]+128)/383;patch([0 1 1 0],[0 0 1 1],c1);patch([0 1 1 1-e 1-e 0+e],[0 0 1 1-e 0+e 0+e],c2);patch([0 0 1 1-e 0+e 0+e],[0 1 1 1-e 1-e 0+e],c3);plot([0 1 1 0 0],[0 0 1 1 0]);disp('weights');
  "IW{2,1}(531,:)'" : Constant  Value=[-1.0707983780938581386266150730079971253871917724609375;0.300120741161163995247562752410885877907276153564453125;1.472316535279533322722045340924523770809173583984375;-0.80561141635986388553902770581771619617938995361328125;0.0231573712683233630393875301933803712017834186553955078125;-1.6947111549094409088667134710703976452350616455078125;-1.8707552847330408685166958093759603798389434814453125;-0.79435652621626184899383815718465484678745269775390625]
      mask Display: e = 0.06;c1 = [120 150 230]/255;c2 = ([120 150 230]+0)/383;c3 = ([120 150 230]+128)/383;patch([0 1 1 0],[0 0 1 1],c1);patch([0 1 1 1-e 1-e 0+e],[0 0 1 1-e 0+e 0+e],c2);patch([0 0 1 1-e 0+e 0+e],[0 1 1 1-e 1-e 0+e],c3);plot([0 1 1 0 0],[0 0 1 1 0]);disp('weights');
  "IW{2,1}(532,:)'" : Constant  Value=[-1.3393050156962311714181623756303451955318450927734375;0.36407714130209445357877484639175236225128173828125;1.3679586287719025516906867778743617236614227294921875;1.428688375248295283626021046075038611888885498046875;1.61061935081682605641617556102573871612548828125;-0.8579326192950491591915351818897761404514312744140625;-0.34842560200630978695102157871588133275508880615234375;1.3128849890910945230615425316500477492809295654296875]
      mask Display: e = 0.06;c1 = [120 150 230]/255;c2 = ([120 150 230]+0)/383;c3 = ([120 150 230]+128)/383;patch([0 1 1 0],[0 0 1 1],c1);patch([0 1 1 1-e 1-e 0+e],[0 0 1 1-e 0+e 0+e],c2);patch([0 0 1 1-e 0+e 0+e],[0 1 1 1-e 1-e 0+e],c3);plot([0 1 1 0 0],[0 0 1 1 0]);disp('weights');
  "IW{2,1}(533,:)'" : Constant  Value=[-0.35457824186738362559623283232212997972965240478515625;-1.01698340445851709290536746266297996044158935546875;-0.6368284515034847714787247241474688053131103515625;1.2801234036670334770491308518103323876857757568359375;-2.34720207759839194494588809902779757976531982421875;0.50795465983103882390281569314538501203060150146484375;1.03163679414547004853375256061553955078125;-0.9721434611444930151691323771956376731395721435546875]
      mask Display: e = 0.06;c1 = [120 150 230]/255;c2 = ([120 150 230]+0)/383;c3 = ([120 150 230]+128)/383;patch([0 1 1 0],[0 0 1 1],c1);patch([0 1 1 1-e 1-e 0+e],[0 0 1 1-e 0+e 0+e],c2);patch([0 0 1 1-e 0+e 0+e],[0 1 1 1-e 1-e 0+e],c3);plot([0 1 1 0 0],[0 0 1 1 0]);disp('weights');
  "IW{2,1}(534,:)'" : Constant  Value=[-1.076316269351698107215042909956537187099456787109375;-1.4952767671908822055826249197707511484622955322265625;-1.0979380208559248455202350669424049556255340576171875;-1.8145886828086918995950327371247112751007080078125;1.606786746745969995942004970856942236423492431640625;0.347805881556428275747094858161290176212787628173828125;0.2423974686110849929843169547893921844661235809326171875;-0.5554202001268875310557859847904182970523834228515625]
      mask Display: e = 0.06;c1 = [120 150 230]/255;c2 = ([120 150 230]+0)/383;c3 = ([120 150 230]+128)/383;patch([0 1 1 0],[0 0 1 1],c1);patch([0 1 1 1-e 1-e 0+e],[0 0 1 1-e 0+e 0+e],c2);patch([0 0 1 1-e 0+e 0+e],[0 1 1 1-e 1-e 0+e],c3);plot([0 1 1 0 0],[0 0 1 1 0]);disp('weights');
  "IW{2,1}(535,:)'" : Constant  Value=[1.73113709470688181824016282917000353336334228515625;-1.32810243899869373507272030110470950603485107421875;-0.03345242100933805418083721860966761596500873565673828125;-0.90269227621514447346129372817813418805599212646484375;-0.364078027872036524836829585183295421302318572998046875;1.4291842879381146946826675048214383423328399658203125;1.357194776012082382266044078278355300426483154296875;1.2005376423315297085281372346798889338970184326171875]
      mask Display: e = 0.06;c1 = [120 150 230]/255;c2 = ([120 150 230]+0)/383;c3 = ([120 150 230]+128)/383;patch([0 1 1 0],[0 0 1 1],c1);patch([0 1 1 1-e 1-e 0+e],[0 0 1 1-e 0+e 0+e],c2);patch([0 0 1 1-e 0+e 0+e],[0 1 1 1-e 1-e 0+e],c3);plot([0 1 1 0 0],[0 0 1 1 0]);disp('weights');
  "IW{2,1}(536,:)'" : Constant  Value=[0.7622347574694485761170881232828833162784576416015625;-1.28951277192080748790203870157711207866668701171875;1.6899745527976843817441476858220994472503662109375;0.761712727951007639859426490147598087787628173828125;-1.7218477765414441638114340094034560024738311767578125;0.57998795054941132409709325656876899302005767822265625;0.82086291862069493685538645877386443316936492919921875;-1.1841652922615757415059078994090668857097625732421875]
      mask Display: e = 0.06;c1 = [120 150 230]/255;c2 = ([120 150 230]+0)/383;c3 = ([120 150 230]+128)/383;patch([0 1 1 0],[0 0 1 1],c1);patch([0 1 1 1-e 1-e 0+e],[0 0 1 1-e 0+e 0+e],c2);patch([0 0 1 1-e 0+e 0+e],[0 1 1 1-e 1-e 0+e],c3);plot([0 1 1 0 0],[0 0 1 1 0]);disp('weights');
  "IW{2,1}(537,:)'" : Constant  Value=[-0.6967548574711390774183428220567293465137481689453125;1.6861531904625890465609927559853531420230865478515625;0.83032599783754712507999329318408854305744171142578125;1.30426626020912550529828877188265323638916015625;-0.791666180129068752790999496937729418277740478515625;-0.619766991825306146068896850920282304286956787109375;1.6714275233778710383347743118065409362316131591796875;-1.2240973371830221605449651178787462413311004638671875]
      mask Display: e = 0.06;c1 = [120 150 230]/255;c2 = ([120 150 230]+0)/383;c3 = ([120 150 230]+128)/383;patch([0 1 1 0],[0 0 1 1],c1);patch([0 1 1 1-e 1-e 0+e],[0 0 1 1-e 0+e 0+e],c2);patch([0 0 1 1-e 0+e 0+e],[0 1 1 1-e 1-e 0+e],c3);plot([0 1 1 0 0],[0 0 1 1 0]);disp('weights');
  "IW{2,1}(538,:)'" : Constant  Value=[-0.81141699225313035359619107111939229071140289306640625;1.894012843808230872610920414444990456104278564453125;0.0200487061927484278012201457386254332959651947021484375;-1.276702760151015692002829382545314729213714599609375;0.464485742048578231777611335928668268024921417236328125;1.0392768581998155230650127123226411640644073486328125;1.9370402424597383816973206194234080612659454345703125;-0.0285621010255329987881367515001329593360424041748046875]
      mask Display: e = 0.06;c1 = [120 150 230]/255;c2 = ([120 150 230]+0)/383;c3 = ([120 150 230]+128)/383;patch([0 1 1 0],[0 0 1 1],c1);patch([0 1 1 1-e 1-e 0+e],[0 0 1 1-e 0+e 0+e],c2);patch([0 0 1 1-e 0+e 0+e],[0 1 1 1-e 1-e 0+e],c3);plot([0 1 1 0 0],[0 0 1 1 0]);disp('weights');
  "IW{2,1}(539,:)'" : Constant  Value=[0.7171190176063866328348694878513924777507781982421875;0.57413612761171928244863238433026708662509918212890625;0.115781342342517745702679121677647344768047332763671875;1.7361299804113310418784976718598045408725738525390625;0.8117168384255666335747037010150961577892303466796875;-1.5654749510795016309572247337200678884983062744140625;-0.92457627136132070067020549686276353895664215087890625;1.834482722015195133025144968996755778789520263671875]
      mask Display: e = 0.06;c1 = [120 150 230]/255;c2 = ([120 150 230]+0)/383;c3 = ([120 150 230]+128)/383;patch([0 1 1 0],[0 0 1 1],c1);patch([0 1 1 1-e 1-e 0+e],[0 0 1 1-e 0+e 0+e],c2);patch([0 0 1 1-e 0+e 0+e],[0 1 1 1-e 1-e 0+e],c3);plot([0 1 1 0 0],[0 0 1 1 0]);disp('weights');
  "IW{2,1}(54,:)'" : Constant  Value=[-0.242597107567060044086559855713858269155025482177734375;-1.3647078044780454053608309550327248871326446533203125;-1.222473562128665758308443400892429053783416748046875;-1.795558410919827707630247459746897220611572265625;1.642538821342431010208429142949171364307403564453125;-1.3478532273227841198348642137716524302959442138671875;-0.296500368958965865306964815317769534885883331298828125;0.08751172773336650390074709093823912553489208221435546875]
      mask Display: e = 0.06;c1 = [120 150 230]/255;c2 = ([120 150 230]+0)/383;c3 = ([120 150 230]+128)/383;patch([0 1 1 0],[0 0 1 1],c1);patch([0 1 1 1-e 1-e 0+e],[0 0 1 1-e 0+e 0+e],c2);patch([0 0 1 1-e 0+e 0+e],[0 1 1 1-e 1-e 0+e],c3);plot([0 1 1 0 0],[0 0 1 1 0]);disp('weights');
  "IW{2,1}(540,:)'" : Constant  Value=[1.4890407420071050115240041122888214886188507080078125;-2.0106564707246423751030306448228657245635986328125;-1.3276789342399322180199305876158177852630615234375;0.92511951120579294371992773449164815247058868408203125;-0.2337137950467539082577417275388143025338649749755859375;-0.4879805867833517663001430264557711780071258544921875;1.129324427523701768194541728007607161998748779296875;0.4021906919344060415966168875456787645816802978515625]
      mask Display: e = 0.06;c1 = [120 150 230]/255;c2 = ([120 150 230]+0)/383;c3 = ([120 150 230]+128)/383;patch([0 1 1 0],[0 0 1 1],c1);patch([0 1 1 1-e 1-e 0+e],[0 0 1 1-e 0+e 0+e],c2);patch([0 0 1 1-e 0+e 0+e],[0 1 1 1-e 1-e 0+e],c3);plot([0 1 1 0 0],[0 0 1 1 0]);disp('weights');
  "IW{2,1}(541,:)'" : Constant  Value=[-0.89202273872678261579238778722356073558330535888671875;-0.418621496119655656098501594897243194282054901123046875;0.301419635482019054872893093488528393208980560302734375;-2.199359019164623507691658232943154871463775634765625;-1.563735610238897510981814775732345879077911376953125;1.382394751326164961113818208104930818080902099609375;0.38384500243532537755442035631858743727207183837890625;-0.7881891334002955051829530930262990295886993408203125]
      mask Display: e = 0.06;c1 = [120 150 230]/255;c2 = ([120 150 230]+0)/383;c3 = ([120 150 230]+128)/383;patch([0 1 1 0],[0 0 1 1],c1);patch([0 1 1 1-e 1-e 0+e],[0 0 1 1-e 0+e 0+e],c2);patch([0 0 1 1-e 0+e 0+e],[0 1 1 1-e 1-e 0+e],c3);plot([0 1 1 0 0],[0 0 1 1 0]);disp('weights');
  "IW{2,1}(542,:)'" : Constant  Value=[0.92181606141338601201340452462318353354930877685546875;1.438438390915918407841900261701084673404693603515625;-0.87138065637195605273035425852867774665355682373046875;1.5491881377924336948836980809574015438556671142578125;1.5697935616055798124790499059599824249744415283203125;0.51161400505914489400538514018990099430084228515625;-0.99563919373017062408592892097658477723598480224609375;-1.1204753966372520412875246620387770235538482666015625]
      mask Display: e = 0.06;c1 = [120 150 230]/255;c2 = ([120 150 230]+0)/383;c3 = ([120 150 230]+128)/383;patch([0 1 1 0],[0 0 1 1],c1);patch([0 1 1 1-e 1-e 0+e],[0 0 1 1-e 0+e 0+e],c2);patch([0 0 1 1-e 0+e 0+e],[0 1 1 1-e 1-e 0+e],c3);plot([0 1 1 0 0],[0 0 1 1 0]);disp('weights');
  "IW{2,1}(543,:)'" : Constant  Value=[-1.4162411257862228541881677301716990768909454345703125;-0.5788542312631108632814402881194837391376495361328125;0.99753548585536189197142675766372121870517730712890625;0.497140070613766915652576017237151972949504852294921875;-2.21231682383596872654152321047149598598480224609375;0.830838794802799984751118245185352861881256103515625;-0.300555183870372999432873939440469257533550262451171875;1.333620811717053822320622202823869884014129638671875]
      mask Display: e = 0.06;c1 = [120 150 230]/255;c2 = ([120 150 230]+0)/383;c3 = ([120 150 230]+128)/383;patch([0 1 1 0],[0 0 1 1],c1);patch([0 1 1 1-e 1-e 0+e],[0 0 1 1-e 0+e 0+e],c2);patch([0 0 1 1-e 0+e 0+e],[0 1 1 1-e 1-e 0+e],c3);plot([0 1 1 0 0],[0 0 1 1 0]);disp('weights');
  "IW{2,1}(544,:)'" : Constant  Value=[0.5283256574928028026505444358917884528636932373046875;1.2769519431100613271468091625138185918331146240234375;-0.1547251044133615416331650749270920641720294952392578125;2.280961455984190866530525454436428844928741455078125;-1.0386210976012006934610099051496945321559906005859375;-0.8100258413158296644240863315644674003124237060546875;1.2875324493939166448086552918539382517337799072265625;0.6973317372321268248214209961588494479656219482421875]
      mask Display: e = 0.06;c1 = [120 150 230]/255;c2 = ([120 150 230]+0)/383;c3 = ([120 150 230]+128)/383;patch([0 1 1 0],[0 0 1 1],c1);patch([0 1 1 1-e 1-e 0+e],[0 0 1 1-e 0+e 0+e],c2);patch([0 0 1 1-e 0+e 0+e],[0 1 1 1-e 1-e 0+e],c3);plot([0 1 1 0 0],[0 0 1 1 0]);disp('weights');
  "IW{2,1}(545,:)'" : Constant  Value=[-0.8239484773400673756071910247555933892726898193359375;-1.810899751470959273547123302705585956573486328125;1.623578898462521014067760916077531874179840087890625;-0.35520248221444827851911441030097194015979766845703125;1.189842076471556264749551701243035495281219482421875;-1.522592454843821219157007362809963524341583251953125;0.33682094946309060201627971764537505805492401123046875;0.67953536524554258857477861965890042483806610107421875]
      mask Display: e = 0.06;c1 = [120 150 230]/255;c2 = ([120 150 230]+0)/383;c3 = ([120 150 230]+128)/383;patch([0 1 1 0],[0 0 1 1],c1);patch([0 1 1 1-e 1-e 0+e],[0 0 1 1-e 0+e 0+e],c2);patch([0 0 1 1-e 0+e 0+e],[0 1 1 1-e 1-e 0+e],c3);plot([0 1 1 0 0],[0 0 1 1 0]);disp('weights');
  "IW{2,1}(546,:)'" : Constant  Value=[0.53288598637495443455236454610712826251983642578125;1.0253433168047718648807631325325928628444671630859375;0.603211308248618127691997869987972080707550048828125;-0.350900797790060503533737801262759603559970855712890625;-1.4373276549503508636718152047251351177692413330078125;-1.3215687087471243987835123334662057459354400634765625;-1.697852908562091922561876344843767583370208740234375;-1.563562055827691921194855240173637866973876953125]
      mask Display: e = 0.06;c1 = [120 150 230]/255;c2 = ([120 150 230]+0)/383;c3 = ([120 150 230]+128)/383;patch([0 1 1 0],[0 0 1 1],c1);patch([0 1 1 1-e 1-e 0+e],[0 0 1 1-e 0+e 0+e],c2);patch([0 0 1 1-e 0+e 0+e],[0 1 1 1-e 1-e 0+e],c3);plot([0 1 1 0 0],[0 0 1 1 0]);disp('weights');
  "IW{2,1}(547,:)'" : Constant  Value=[0.7625335798226309247382914691115729510784149169921875;1.279940745199312335245167560060508549213409423828125;-0.6343186683095638489504608514835126698017120361328125;1.310280977446467431946075521409511566162109375;-1.5844533798915787503602814467740245163440704345703125;1.5074527443454908137709935544990003108978271484375;-1.3093895277364888674043186256312765181064605712890625;0.43742574796708810769274577978649176657199859619140625]
      mask Display: e = 0.06;c1 = [120 150 230]/255;c2 = ([120 150 230]+0)/383;c3 = ([120 150 230]+128)/383;patch([0 1 1 0],[0 0 1 1],c1);patch([0 1 1 1-e 1-e 0+e],[0 0 1 1-e 0+e 0+e],c2);patch([0 0 1 1-e 0+e 0+e],[0 1 1 1-e 1-e 0+e],c3);plot([0 1 1 0 0],[0 0 1 1 0]);disp('weights');
  "IW{2,1}(548,:)'" : Constant  Value=[0.315051130892553932216770817831275053322315216064453125;1.1993642826531651923716026431065984070301055908203125;0.64716451919116113611352147927391342818737030029296875;-1.15349535580205309059920182335190474987030029296875;-1.1968261481308497540254620616906322538852691650390625;0.319527526158513153209383972352952696382999420166015625;1.07529025165320835100146723561920225620269775390625;-2.21887243304556847078856662847101688385009765625]
      mask Display: e = 0.06;c1 = [120 150 230]/255;c2 = ([120 150 230]+0)/383;c3 = ([120 150 230]+128)/383;patch([0 1 1 0],[0 0 1 1],c1);patch([0 1 1 1-e 1-e 0+e],[0 0 1 1-e 0+e 0+e],c2);patch([0 0 1 1-e 0+e 0+e],[0 1 1 1-e 1-e 0+e],c3);plot([0 1 1 0 0],[0 0 1 1 0]);disp('weights');
  "IW{2,1}(549,:)'" : Constant  Value=[-1.2114377907713149706836475161253474652767181396484375;-1.0819335077601952566084264617529697716236114501953125;-1.5957023612419376501492251918534748256206512451171875;0.95552475822940563521257217871607281267642974853515625;0.8787623068911607493447490924154408276081085205078125;-0.960957776343674741070799427689053118228912353515625;0.50309421600879777880521714905626140534877777099609375;-1.7533635004316481253994197686552070081233978271484375]
      mask Display: e = 0.06;c1 = [120 150 230]/255;c2 = ([120 150 230]+0)/383;c3 = ([120 150 230]+128)/383;patch([0 1 1 0],[0 0 1 1],c1);patch([0 1 1 1-e 1-e 0+e],[0 0 1 1-e 0+e 0+e],c2);patch([0 0 1 1-e 0+e 0+e],[0 1 1 1-e 1-e 0+e],c3);plot([0 1 1 0 0],[0 0 1 1 0]);disp('weights');
  "IW{2,1}(55,:)'" : Constant  Value=[-0.0063190148238002098735055511724567622877657413482666015625;-1.232866839213078602455198051757179200649261474609375;1.4915319838355574066923736609169282019138336181640625;-0.646963822194997373316027733380906283855438232421875;-1.6240251095114384138895502474042586982250213623046875;0.9740185017194058492151498285238631069660186767578125;-0.86131853569624905464507946817320771515369415283203125;1.590274546343668049530606367625296115875244140625]
      mask Display: e = 0.06;c1 = [120 150 230]/255;c2 = ([120 150 230]+0)/383;c3 = ([120 150 230]+128)/383;patch([0 1 1 0],[0 0 1 1],c1);patch([0 1 1 1-e 1-e 0+e],[0 0 1 1-e 0+e 0+e],c2);patch([0 0 1 1-e 0+e 0+e],[0 1 1 1-e 1-e 0+e],c3);plot([0 1 1 0 0],[0 0 1 1 0]);disp('weights');
  "IW{2,1}(550,:)'" : Constant  Value=[0.99765371358831800296940173211623914539813995361328125;-0.75834213273457951043354796638595871627330780029296875;1.518420050234954743473281268961727619171142578125;-0.9306852074970939359133126345113851130008697509765625;0.83627148572161846828976194956339895725250244140625;-1.6783307405672343026736825777334161102771759033203125;0.567692246776750675252287692273966968059539794921875;1.5680516547934886251169928073068149387836456298828125]
      mask Display: e = 0.06;c1 = [120 150 230]/255;c2 = ([120 150 230]+0)/383;c3 = ([120 150 230]+128)/383;patch([0 1 1 0],[0 0 1 1],c1);patch([0 1 1 1-e 1-e 0+e],[0 0 1 1-e 0+e 0+e],c2);patch([0 0 1 1-e 0+e 0+e],[0 1 1 1-e 1-e 0+e],c3);plot([0 1 1 0 0],[0 0 1 1 0]);disp('weights');
  "IW{2,1}(551,:)'" : Constant  Value=[0.2482831348297062923347056084821815602481365203857421875;-0.342391536293973952620461886908742599189281463623046875;-0.69499063872623201287836991468793712556362152099609375;1.658067076217502933133118858677335083484649658203125;0.69592512987843224703254918495076708495616912841796875;-1.8380285705556798081516944876057095825672149658203125;1.5141782634737717128103895447566173970699310302734375;-1.2366556645098840672147844088613055646419525146484375]
      mask Display: e = 0.06;c1 = [120 150 230]/255;c2 = ([120 150 230]+0)/383;c3 = ([120 150 230]+128)/383;patch([0 1 1 0],[0 0 1 1],c1);patch([0 1 1 1-e 1-e 0+e],[0 0 1 1-e 0+e 0+e],c2);patch([0 0 1 1-e 0+e 0+e],[0 1 1 1-e 1-e 0+e],c3);plot([0 1 1 0 0],[0 0 1 1 0]);disp('weights');
  "IW{2,1}(552,:)'" : Constant  Value=[1.6183721892476958803541720044449903070926666259765625;-0.38932902856502715760456112548126839101314544677734375;-0.5196550490021645263283289750688709318637847900390625;0.944596491035306851102859582169912755489349365234375;1.288202376844671537270414773956872522830963134765625;-1.5180041990022539177829230538918636739253997802734375;1.2463443925290202951572382517042569816112518310546875;1.2526564090334684209437909885309636592864990234375]
      mask Display: e = 0.06;c1 = [120 150 230]/255;c2 = ([120 150 230]+0)/383;c3 = ([120 150 230]+128)/383;patch([0 1 1 0],[0 0 1 1],c1);patch([0 1 1 1-e 1-e 0+e],[0 0 1 1-e 0+e 0+e],c2);patch([0 0 1 1-e 0+e 0+e],[0 1 1 1-e 1-e 0+e],c3);plot([0 1 1 0 0],[0 0 1 1 0]);disp('weights');
  "IW{2,1}(553,:)'" : Constant  Value=[0.168237147724541402649123256196617148816585540771484375;-1.4586116932604131779527278922614641487598419189453125;-1.5510219291188171997220024422858841717243194580078125;1.74095902277251912693145641242153942584991455078125;-1.632288940821168043981970185996033251285552978515625;0.88608587954818063270323591495980508625507354736328125;-0.1599106908455759923359806862208642996847629547119140625;0.036035864759457685024823803132676403038203716278076171875]
      mask Display: e = 0.06;c1 = [120 150 230]/255;c2 = ([120 150 230]+0)/383;c3 = ([120 150 230]+128)/383;patch([0 1 1 0],[0 0 1 1],c1);patch([0 1 1 1-e 1-e 0+e],[0 0 1 1-e 0+e 0+e],c2);patch([0 0 1 1-e 0+e 0+e],[0 1 1 1-e 1-e 0+e],c3);plot([0 1 1 0 0],[0 0 1 1 0]);disp('weights');
  "IW{2,1}(554,:)'" : Constant  Value=[1.1641461288917620553462484167539514601230621337890625;-0.27685661717184750774123358496581204235553741455078125;2.08594249974182144313772369059734046459197998046875;-0.0306034775371246507702505113002189318649470806121826171875;-1.832785523126176929764596934546716511249542236328125;1.1348170147593619194736902500153519213199615478515625;0.4234214379492888813416584525839425623416900634765625;0.61413310114733954403476445804699324071407318115234375]
      mask Display: e = 0.06;c1 = [120 150 230]/255;c2 = ([120 150 230]+0)/383;c3 = ([120 150 230]+128)/383;patch([0 1 1 0],[0 0 1 1],c1);patch([0 1 1 1-e 1-e 0+e],[0 0 1 1-e 0+e 0+e],c2);patch([0 0 1 1-e 0+e 0+e],[0 1 1 1-e 1-e 0+e],c3);plot([0 1 1 0 0],[0 0 1 1 0]);disp('weights');
  "IW{2,1}(555,:)'" : Constant  Value=[1.7483856598286335870540142423124052584171295166015625;-1.61605988321038385180372642935253679752349853515625;1.242260831024060596661229283199645578861236572265625;-1.2480061327460634235109182554879225790500640869140625;0.72363728649682113047703069241833873093128204345703125;0.38104771676248982981149993065628223121166229248046875;-1.042509127823903813947481467039324343204498291015625;0.296276844645128267785594289307482540607452392578125]
      mask Display: e = 0.06;c1 = [120 150 230]/255;c2 = ([120 150 230]+0)/383;c3 = ([120 150 230]+128)/383;patch([0 1 1 0],[0 0 1 1],c1);patch([0 1 1 1-e 1-e 0+e],[0 0 1 1-e 0+e 0+e],c2);patch([0 0 1 1-e 0+e 0+e],[0 1 1 1-e 1-e 0+e],c3);plot([0 1 1 0 0],[0 0 1 1 0]);disp('weights');
  "IW{2,1}(556,:)'" : Constant  Value=[0.94119718457102174991035781204118393361568450927734375;-1.15364921073551318642103069578297436237335205078125;-1.06476637032003029759152923361398279666900634765625;1.4868317122317133982534187452984042465686798095703125;1.5226492671876783457918236308614723384380340576171875;-0.5293062380374868869381543845520354807376861572265625;-1.5650893655013768945849506053491495549678802490234375;-0.594961205986593189010136484284885227680206298828125]
      mask Display: e = 0.06;c1 = [120 150 230]/255;c2 = ([120 150 230]+0)/383;c3 = ([120 150 230]+128)/383;patch([0 1 1 0],[0 0 1 1],c1);patch([0 1 1 1-e 1-e 0+e],[0 0 1 1-e 0+e 0+e],c2);patch([0 0 1 1-e 0+e 0+e],[0 1 1 1-e 1-e 0+e],c3);plot([0 1 1 0 0],[0 0 1 1 0]);disp('weights');
  "IW{2,1}(557,:)'" : Constant  Value=[1.8237870235997404311234504348249174654483795166015625;1.3655030923339472881394840442226268351078033447265625;1.8619721050175517262914581806398928165435791015625;1.000303410970300177496028481982648372650146484375;-1.14743609953859770911321902531199157238006591796875;-0.1111881679567917335926807709256536327302455902099609375;-0.2418154135741842070128626573932706378400325775146484375;0.157443645224574602092815212017740122973918914794921875]
      mask Display: e = 0.06;c1 = [120 150 230]/255;c2 = ([120 150 230]+0)/383;c3 = ([120 150 230]+128)/383;patch([0 1 1 0],[0 0 1 1],c1);patch([0 1 1 1-e 1-e 0+e],[0 0 1 1-e 0+e 0+e],c2);patch([0 0 1 1-e 0+e 0+e],[0 1 1 1-e 1-e 0+e],c3);plot([0 1 1 0 0],[0 0 1 1 0]);disp('weights');
  "IW{2,1}(558,:)'" : Constant  Value=[0.32299700545039533583491220269934274256229400634765625;-0.395741035391215467686976126060471870005130767822265625;-1.27666534148304577911403612233698368072509765625;-1.6994736132454344446074401275836862623691558837890625;-0.0997227065232021148144525568568496964871883392333984375;1.4706692214108729732657820932217873632907867431640625;-0.6163940822423354948256246643722988665103912353515625;-1.88870999594574850988237812998704612255096435546875]
      mask Display: e = 0.06;c1 = [120 150 230]/255;c2 = ([120 150 230]+0)/383;c3 = ([120 150 230]+128)/383;patch([0 1 1 0],[0 0 1 1],c1);patch([0 1 1 1-e 1-e 0+e],[0 0 1 1-e 0+e 0+e],c2);patch([0 0 1 1-e 0+e 0+e],[0 1 1 1-e 1-e 0+e],c3);plot([0 1 1 0 0],[0 0 1 1 0]);disp('weights');
  "IW{2,1}(559,:)'" : Constant  Value=[-1.7917441245491068091411079876706935465335845947265625;0.60900434746063325519571662880480289459228515625;-0.35832040117921926114519237671629525721073150634765625;-1.8204607468044831097842006784048862755298614501953125;-0.9131782825818433035891530380467884242534637451171875;-0.210519485425669838907225539514911361038684844970703125;1.24219235919428516723428401746787130832672119140625;1.22808306075882978092295161332003772258758544921875]
      mask Display: e = 0.06;c1 = [120 150 230]/255;c2 = ([120 150 230]+0)/383;c3 = ([120 150 230]+128)/383;patch([0 1 1 0],[0 0 1 1],c1);patch([0 1 1 1-e 1-e 0+e],[0 0 1 1-e 0+e 0+e],c2);patch([0 0 1 1-e 0+e 0+e],[0 1 1 1-e 1-e 0+e],c3);plot([0 1 1 0 0],[0 0 1 1 0]);disp('weights');
  "IW{2,1}(56,:)'" : Constant  Value=[1.0154333751677324659823398178559727966785430908203125;1.5038205657820074012676059282966889441013336181640625;-1.036903752580653037540514560532756149768829345703125;-0.98354957554064281755046295074862428009510040283203125;0.38671174011299858097601145345834083855152130126953125;0.14485990631778966619691573214367963373661041259765625;-1.51583916284657771456068076076917350292205810546875;-1.79427035702713855158663136535324156284332275390625]
      mask Display: e = 0.06;c1 = [120 150 230]/255;c2 = ([120 150 230]+0)/383;c3 = ([120 150 230]+128)/383;patch([0 1 1 0],[0 0 1 1],c1);patch([0 1 1 1-e 1-e 0+e],[0 0 1 1-e 0+e 0+e],c2);patch([0 0 1 1-e 0+e 0+e],[0 1 1 1-e 1-e 0+e],c3);plot([0 1 1 0 0],[0 0 1 1 0]);disp('weights');
  "IW{2,1}(560,:)'" : Constant  Value=[1.650583131448195128854194990708492696285247802734375;1.3434509372289988871074228882207535207271575927734375;-0.10152524628773869352915681929516722448170185089111328125;0.254724377198585205661629515816457569599151611328125;1.3790250649816264694180745209450833499431610107421875;1.22008728126881305087181317503564059734344482421875;0.60818279667204910854394483976648189127445220947265625;-1.6406457950285109337329458867316134274005889892578125]
      mask Display: e = 0.06;c1 = [120 150 230]/255;c2 = ([120 150 230]+0)/383;c3 = ([120 150 230]+128)/383;patch([0 1 1 0],[0 0 1 1],c1);patch([0 1 1 1-e 1-e 0+e],[0 0 1 1-e 0+e 0+e],c2);patch([0 0 1 1-e 0+e 0+e],[0 1 1 1-e 1-e 0+e],c3);plot([0 1 1 0 0],[0 0 1 1 0]);disp('weights');
  "IW{2,1}(561,:)'" : Constant  Value=[-1.2833300864831522769549110307707451283931732177734375;-0.27917480205423661487884601228870451450347900390625;-0.4055942876237708105691126547753810882568359375;-2.2158408361649097884082948439754545688629150390625;1.7205009378068496506131168644060380756855010986328125;-0.61941302637922246443480389643809758126735687255859375;-0.46921132883364291554784131221822462975978851318359375;-0.799672812022399259745952804223634302616119384765625]
      mask Display: e = 0.06;c1 = [120 150 230]/255;c2 = ([120 150 230]+0)/383;c3 = ([120 150 230]+128)/383;patch([0 1 1 0],[0 0 1 1],c1);patch([0 1 1 1-e 1-e 0+e],[0 0 1 1-e 0+e 0+e],c2);patch([0 0 1 1-e 0+e 0+e],[0 1 1 1-e 1-e 0+e],c3);plot([0 1 1 0 0],[0 0 1 1 0]);disp('weights');
  "IW{2,1}(562,:)'" : Constant  Value=[-1.78822709304308258282389942905865609645843505859375;1.30629709862651122165289052645675837993621826171875;-1.02150022101226767290427233092486858367919921875;0.24829031266287426849004305040580220520496368408203125;-1.136885992641607945330406437278725206851959228515625;-0.6155240024445955970833210812998004257678985595703125;-0.277920777267101792862291631536209024488925933837890625;-1.810286685369329351402711836271919310092926025390625]
      mask Display: e = 0.06;c1 = [120 150 230]/255;c2 = ([120 150 230]+0)/383;c3 = ([120 150 230]+128)/383;patch([0 1 1 0],[0 0 1 1],c1);patch([0 1 1 1-e 1-e 0+e],[0 0 1 1-e 0+e 0+e],c2);patch([0 0 1 1-e 0+e 0+e],[0 1 1 1-e 1-e 0+e],c3);plot([0 1 1 0 0],[0 0 1 1 0]);disp('weights');
  "IW{2,1}(563,:)'" : Constant  Value=[-1.412123530235021906520387346972711384296417236328125;-1.3699936706060735769341363265994004905223846435546875;0.88206500374061003189041230143629945814609527587890625;-1.5801989858556544366052776240394450724124908447265625;0.607685879592450906017120360047556459903717041015625;-0.68899889579764650449078544625081121921539306640625;1.5739731211626912799061983605497516691684722900390625;-0.705846253338181295333697562455199658870697021484375]
      mask Display: e = 0.06;c1 = [120 150 230]/255;c2 = ([120 150 230]+0)/383;c3 = ([120 150 230]+128)/383;patch([0 1 1 0],[0 0 1 1],c1);patch([0 1 1 1-e 1-e 0+e],[0 0 1 1-e 0+e 0+e],c2);patch([0 0 1 1-e 0+e 0+e],[0 1 1 1-e 1-e 0+e],c3);plot([0 1 1 0 0],[0 0 1 1 0]);disp('weights');
  "IW{2,1}(564,:)'" : Constant  Value=[-0.31456761178804215628446172559051774442195892333984375;0.02663418902394083798146340313905966468155384063720703125;0.225039666291946272025370490155182778835296630859375;-0.11833562966615097933331668400569469667971134185791015625;-0.30410759403486065099997404104215092957019805908203125;-2.27500510260892685465705653768964111804962158203125;1.9579136794826508261024855528376065194606781005859375;1.249257776695452459847501813783310353755950927734375]
      mask Display: e = 0.06;c1 = [120 150 230]/255;c2 = ([120 150 230]+0)/383;c3 = ([120 150 230]+128)/383;patch([0 1 1 0],[0 0 1 1],c1);patch([0 1 1 1-e 1-e 0+e],[0 0 1 1-e 0+e 0+e],c2);patch([0 0 1 1-e 0+e 0+e],[0 1 1 1-e 1-e 0+e],c3);plot([0 1 1 0 0],[0 0 1 1 0]);disp('weights');
  "IW{2,1}(565,:)'" : Constant  Value=[0.465427484740867647428075315474416129291057586669921875;1.2096801823287448574006930357427336275577545166015625;0.64775344939490320239627862974884919822216033935546875;-1.508587463000045314487351788557134568691253662109375;-1.465617188506477486242829399998299777507781982421875;1.570009032887816236012668014154769480228424072265625;-0.646719147399569482814740695175714790821075439453125;1.2371501156205180205205351740005426108837127685546875]
      mask Display: e = 0.06;c1 = [120 150 230]/255;c2 = ([120 150 230]+0)/383;c3 = ([120 150 230]+128)/383;patch([0 1 1 0],[0 0 1 1],c1);patch([0 1 1 1-e 1-e 0+e],[0 0 1 1-e 0+e 0+e],c2);patch([0 0 1 1-e 0+e 0+e],[0 1 1 1-e 1-e 0+e],c3);plot([0 1 1 0 0],[0 0 1 1 0]);disp('weights');
  "IW{2,1}(566,:)'" : Constant  Value=[-0.8789292606901064619506769304280169308185577392578125;1.3275167414195205850546699366532266139984130859375;1.0373556960749030775303936025011353194713592529296875;-1.0644354681092977887857387031544931232929229736328125;1.687360738047574582054721759050153195858001708984375;-0.340016575974306844987182785189361311495304107666015625;0.70909660303447641371832332879421301186084747314453125;-1.7049127690600911488871815890888683497905731201171875]
      mask Display: e = 0.06;c1 = [120 150 230]/255;c2 = ([120 150 230]+0)/383;c3 = ([120 150 230]+128)/383;patch([0 1 1 0],[0 0 1 1],c1);patch([0 1 1 1-e 1-e 0+e],[0 0 1 1-e 0+e 0+e],c2);patch([0 0 1 1-e 0+e 0+e],[0 1 1 1-e 1-e 0+e],c3);plot([0 1 1 0 0],[0 0 1 1 0]);disp('weights');
  "IW{2,1}(567,:)'" : Constant  Value=[-0.3300734455038860648556919841212220489978790283203125;-0.94935643394856350507637898772372864186763763427734375;-1.3786132445261458645546781554003246128559112548828125;-0.9761777641369560054585008401772938668727874755859375;1.7137733031677819806049001272185705602169036865234375;1.08420942820541998941052952432073652744293212890625;1.781489625251493347235509645543061196804046630859375;0.10652014410866779414721605689919670112431049346923828125]
      mask Display: e = 0.06;c1 = [120 150 230]/255;c2 = ([120 150 230]+0)/383;c3 = ([120 150 230]+128)/383;patch([0 1 1 0],[0 0 1 1],c1);patch([0 1 1 1-e 1-e 0+e],[0 0 1 1-e 0+e 0+e],c2);patch([0 0 1 1-e 0+e 0+e],[0 1 1 1-e 1-e 0+e],c3);plot([0 1 1 0 0],[0 0 1 1 0]);disp('weights');
  "IW{2,1}(568,:)'" : Constant  Value=[-0.351580894744753125191749631994753144681453704833984375;1.648834671587044109486441811895929276943206787109375;0.10362198187780051472639541998432832770049571990966796875;1.4033762166806520443884664928191341459751129150390625;-0.9641201236610612568256328813731670379638671875;-1.6515784586491399910102018111501820385456085205078125;0.2809010419200195229905148153193295001983642578125;1.6235797567389571582907592528499662876129150390625]
      mask Display: e = 0.06;c1 = [120 150 230]/255;c2 = ([120 150 230]+0)/383;c3 = ([120 150 230]+128)/383;patch([0 1 1 0],[0 0 1 1],c1);patch([0 1 1 1-e 1-e 0+e],[0 0 1 1-e 0+e 0+e],c2);patch([0 0 1 1-e 0+e 0+e],[0 1 1 1-e 1-e 0+e],c3);plot([0 1 1 0 0],[0 0 1 1 0]);disp('weights');
  "IW{2,1}(569,:)'" : Constant  Value=[0.7324949117401953202488584793172776699066162109375;1.1811814086798804179778699108283035457134246826171875;0.73040750812838883820887758702156133949756622314453125;-1.23257604620489136237893035286106169223785400390625;1.22262672055779564317390395444817841053009033203125;-0.7696373410468011488916317830444313585758209228515625;-1.7470033674548848257046529397484846413135528564453125;-1.503423577235053709699741375516168773174285888671875]
      mask Display: e = 0.06;c1 = [120 150 230]/255;c2 = ([120 150 230]+0)/383;c3 = ([120 150 230]+128)/383;patch([0 1 1 0],[0 0 1 1],c1);patch([0 1 1 1-e 1-e 0+e],[0 0 1 1-e 0+e 0+e],c2);patch([0 0 1 1-e 0+e 0+e],[0 1 1 1-e 1-e 0+e],c3);plot([0 1 1 0 0],[0 0 1 1 0]);disp('weights');
  "IW{2,1}(57,:)'" : Constant  Value=[-1.1672634589275292515964110862114466726779937744140625;1.6497046723973285420328238615184091031551361083984375;-0.337786867311482164044633691446506418287754058837890625;1.5746958725383766175554001165437512099742889404296875;0.88177975150395682124582208416541106998920440673828125;1.5379880871788731422356022449093870818614959716796875;0.9034002969510017688747893771505914628505706787109375;-0.61785358790772326731399743948713876307010650634765625]
      mask Display: e = 0.06;c1 = [120 150 230]/255;c2 = ([120 150 230]+0)/383;c3 = ([120 150 230]+128)/383;patch([0 1 1 0],[0 0 1 1],c1);patch([0 1 1 1-e 1-e 0+e],[0 0 1 1-e 0+e 0+e],c2);patch([0 0 1 1-e 0+e 0+e],[0 1 1 1-e 1-e 0+e],c3);plot([0 1 1 0 0],[0 0 1 1 0]);disp('weights');
  "IW{2,1}(570,:)'" : Constant  Value=[-1.7608105790623671538241978851146996021270751953125;0.9079964836773160019589568037190474569797515869140625;-0.97421802889136632774835788950440473854541778564453125;0.63723036190987680793540448576095513999462127685546875;0.396791505054111592887267079277080483734607696533203125;1.3956769854762012261772952115279622375965118408203125;-1.8665520301770353039927385907503776252269744873046875;-0.479654259527794835094027803279459476470947265625]
      mask Display: e = 0.06;c1 = [120 150 230]/255;c2 = ([120 150 230]+0)/383;c3 = ([120 150 230]+128)/383;patch([0 1 1 0],[0 0 1 1],c1);patch([0 1 1 1-e 1-e 0+e],[0 0 1 1-e 0+e 0+e],c2);patch([0 0 1 1-e 0+e 0+e],[0 1 1 1-e 1-e 0+e],c3);plot([0 1 1 0 0],[0 0 1 1 0]);disp('weights');
  "IW{2,1}(571,:)'" : Constant  Value=[1.261549966905576081188655734877102077007293701171875;0.941542033159857627566680093877948820590972900390625;-1.328151023309118272663909010589122772216796875;1.211360414599301993376911923405714333057403564453125;-1.151728177337826508619400556199252605438232421875;-1.3199449352670582502611296149552799761295318603515625;0.31979724863217418029393002143478952348232269287109375;1.39128562127888244503992609679698944091796875]
      mask Display: e = 0.06;c1 = [120 150 230]/255;c2 = ([120 150 230]+0)/383;c3 = ([120 150 230]+128)/383;patch([0 1 1 0],[0 0 1 1],c1);patch([0 1 1 1-e 1-e 0+e],[0 0 1 1-e 0+e 0+e],c2);patch([0 0 1 1-e 0+e 0+e],[0 1 1 1-e 1-e 0+e],c3);plot([0 1 1 0 0],[0 0 1 1 0]);disp('weights');
  "IW{2,1}(572,:)'" : Constant  Value=[-1.322637874594189799637433679890818893909454345703125;-1.932051177446947765048435030621476471424102783203125;0.485384198640600394991651000964338891208171844482421875;0.345045923025805001405075245202169753611087799072265625;0.67443639395410237558081689712707884609699249267578125;-0.477909299037757973049878046367666684091091156005859375;2.071987058300726491921750493929721415042877197265625;-0.35035275330851500807938236903282813727855682373046875]
      mask Display: e = 0.06;c1 = [120 150 230]/255;c2 = ([120 150 230]+0)/383;c3 = ([120 150 230]+128)/383;patch([0 1 1 0],[0 0 1 1],c1);patch([0 1 1 1-e 1-e 0+e],[0 0 1 1-e 0+e 0+e],c2);patch([0 0 1 1-e 0+e 0+e],[0 1 1 1-e 1-e 0+e],c3);plot([0 1 1 0 0],[0 0 1 1 0]);disp('weights');
  "IW{2,1}(573,:)'" : Constant  Value=[-0.51903313297773812085011968520120717585086822509765625;1.25140261911566863517464298638515174388885498046875;-0.2807038339437559759659279734478332102298736572265625;-0.83486714961524477462972981811617501080036163330078125;-1.5131361239134222262947560011525638401508331298828125;2.15560248831752421239116301876492798328399658203125;-0.11566530820758076647525314228914794512093067169189453125;-1.256237681213635770660630441852845251560211181640625]
      mask Display: e = 0.06;c1 = [120 150 230]/255;c2 = ([120 150 230]+0)/383;c3 = ([120 150 230]+128)/383;patch([0 1 1 0],[0 0 1 1],c1);patch([0 1 1 1-e 1-e 0+e],[0 0 1 1-e 0+e 0+e],c2);patch([0 0 1 1-e 0+e 0+e],[0 1 1 1-e 1-e 0+e],c3);plot([0 1 1 0 0],[0 0 1 1 0]);disp('weights');
  "IW{2,1}(574,:)'" : Constant  Value=[-0.745944192672386208187162992544472217559814453125;1.398352626629705497407485381700098514556884765625;1.3480192068268250782381301178247667849063873291015625;-1.870638532185445956912417386774905025959014892578125;-1.1209688903491252798261257339618168771266937255859375;-0.40069793418299715082042666836059652268886566162109375;-1.2798784495783424031145614208071492612361907958984375;-0.374068192426130707861631208288599736988544464111328125]
      mask Display: e = 0.06;c1 = [120 150 230]/255;c2 = ([120 150 230]+0)/383;c3 = ([120 150 230]+128)/383;patch([0 1 1 0],[0 0 1 1],c1);patch([0 1 1 1-e 1-e 0+e],[0 0 1 1-e 0+e 0+e],c2);patch([0 0 1 1-e 0+e 0+e],[0 1 1 1-e 1-e 0+e],c3);plot([0 1 1 0 0],[0 0 1 1 0]);disp('weights');
  "IW{2,1}(575,:)'" : Constant  Value=[-0.51969151623279452589798665940179489552974700927734375;0.93910834716368840613398560890345834195613861083984375;0.89737617785034495820895017459406517446041107177734375;1.313694724451334838732918797177262604236602783203125;0.62316406285131531461729537113569676876068115234375;1.7818803484022118777119203514303080737590789794921875;-1.259287580493402725068108338746242225170135498046875;1.52522822474873631648506489000283181667327880859375]
      mask Display: e = 0.06;c1 = [120 150 230]/255;c2 = ([120 150 230]+0)/383;c3 = ([120 150 230]+128)/383;patch([0 1 1 0],[0 0 1 1],c1);patch([0 1 1 1-e 1-e 0+e],[0 0 1 1-e 0+e 0+e],c2);patch([0 0 1 1-e 0+e 0+e],[0 1 1 1-e 1-e 0+e],c3);plot([0 1 1 0 0],[0 0 1 1 0]);disp('weights');
  "IW{2,1}(576,:)'" : Constant  Value=[1.025349526105323594293849964742548763751983642578125;0.358551218764207646483299640749464742839336395263671875;-0.04803348655614748941022895678543136455118656158447265625;0.1462905428733360102544480696451500989496707916259765625;1.817908654371425125617633966612629592418670654296875;1.927840873682816091871927710599265992641448974609375;1.137951111757993682971346061094664037227630615234375;-1.222997891707664042115766278584487736225128173828125]
      mask Display: e = 0.06;c1 = [120 150 230]/255;c2 = ([120 150 230]+0)/383;c3 = ([120 150 230]+128)/383;patch([0 1 1 0],[0 0 1 1],c1);patch([0 1 1 1-e 1-e 0+e],[0 0 1 1-e 0+e 0+e],c2);patch([0 0 1 1-e 0+e 0+e],[0 1 1 1-e 1-e 0+e],c3);plot([0 1 1 0 0],[0 0 1 1 0]);disp('weights');
  "IW{2,1}(577,:)'" : Constant  Value=[-0.95083806538489479276421434406074695289134979248046875;1.0532823914271716159163361226092092692852020263671875;-1.1635706753420149706101938136271201074123382568359375;1.2860463393860361858145324731594882905483245849609375;-1.1666614189833859338563115670694969594478607177734375;-1.3466682386161343831787462477223016321659088134765625;1.12375868854117388906388441682793200016021728515625;-1.2615909916731877782325454973033629357814788818359375]
      mask Display: e = 0.06;c1 = [120 150 230]/255;c2 = ([120 150 230]+0)/383;c3 = ([120 150 230]+128)/383;patch([0 1 1 0],[0 0 1 1],c1);patch([0 1 1 1-e 1-e 0+e],[0 0 1 1-e 0+e 0+e],c2);patch([0 0 1 1-e 0+e 0+e],[0 1 1 1-e 1-e 0+e],c3);plot([0 1 1 0 0],[0 0 1 1 0]);disp('weights');
  "IW{2,1}(578,:)'" : Constant  Value=[1.923726661204394172699494447442702949047088623046875;0.48963149066955591326433250287664122879505157470703125;-0.230544243297397255521019587831688113510608673095703125;-0.99429985145689092629339711493230424821376800537109375;-0.9520788264181903048921640220214612782001495361328125;1.641254360166387815667121685692109167575836181640625;1.3405157759586801002882339162169955670833587646484375;-0.77788545675538156576322990076732821762561798095703125]
      mask Display: e = 0.06;c1 = [120 150 230]/255;c2 = ([120 150 230]+0)/383;c3 = ([120 150 230]+128)/383;patch([0 1 1 0],[0 0 1 1],c1);patch([0 1 1 1-e 1-e 0+e],[0 0 1 1-e 0+e 0+e],c2);patch([0 0 1 1-e 0+e 0+e],[0 1 1 1-e 1-e 0+e],c3);plot([0 1 1 0 0],[0 0 1 1 0]);disp('weights');
  "IW{2,1}(579,:)'" : Constant  Value=[0.075381757429366313960628076529246754944324493408203125;-0.5875964170644893957984322696574963629245758056640625;-1.7053692914587401663339960578014142811298370361328125;1.2397088801583275863293920338037423789501190185546875;-0.990845546629215423450887101353146135807037353515625;1.0440954194998053328191645050537772476673126220703125;0.54086439409961106772328776060021482408046722412109375;-2.00048468685362390573345692246221005916595458984375]
      mask Display: e = 0.06;c1 = [120 150 230]/255;c2 = ([120 150 230]+0)/383;c3 = ([120 150 230]+128)/383;patch([0 1 1 0],[0 0 1 1],c1);patch([0 1 1 1-e 1-e 0+e],[0 0 1 1-e 0+e 0+e],c2);patch([0 0 1 1-e 0+e 0+e],[0 1 1 1-e 1-e 0+e],c3);plot([0 1 1 0 0],[0 0 1 1 0]);disp('weights');
  "IW{2,1}(58,:)'" : Constant  Value=[0.8550880174457249349728726883768104016780853271484375;-1.087108801701563987052168158697895705699920654296875;0.370348459155305842482874822962912730872631072998046875;1.7102475684923283960614526222343556582927703857421875;-1.693290145409439784174310261732898652553558349609375;1.46209927201441747257604220067150890827178955078125;-1.0737282273076822480817327232216484844684600830078125;0.20211586383642643482971834600903093814849853515625]
      mask Display: e = 0.06;c1 = [120 150 230]/255;c2 = ([120 150 230]+0)/383;c3 = ([120 150 230]+128)/383;patch([0 1 1 0],[0 0 1 1],c1);patch([0 1 1 1-e 1-e 0+e],[0 0 1 1-e 0+e 0+e],c2);patch([0 0 1 1-e 0+e 0+e],[0 1 1 1-e 1-e 0+e],c3);plot([0 1 1 0 0],[0 0 1 1 0]);disp('weights');
  "IW{2,1}(580,:)'" : Constant  Value=[-1.0003790438202571078107894209097139537334442138671875;-1.391181057452044900202281496603973209857940673828125;0.4769625064284837012706930181593634188175201416015625;1.1649974850860704833621639409102499485015869140625;-1.3976249906065787431685976116568781435489654541015625;-1.1295991618811360712726354904589243233203887939453125;0.46056218231963341747103868328849785029888153076171875;-1.7391218678540198983029085866292007267475128173828125]
      mask Display: e = 0.06;c1 = [120 150 230]/255;c2 = ([120 150 230]+0)/383;c3 = ([120 150 230]+128)/383;patch([0 1 1 0],[0 0 1 1],c1);patch([0 1 1 1-e 1-e 0+e],[0 0 1 1-e 0+e 0+e],c2);patch([0 0 1 1-e 0+e 0+e],[0 1 1 1-e 1-e 0+e],c3);plot([0 1 1 0 0],[0 0 1 1 0]);disp('weights');
  "IW{2,1}(581,:)'" : Constant  Value=[-0.95360053952299972390704851932241581380367279052734375;-1.188706943209054234245058978558517992496490478515625;-1.6144652761466300461279388400726020336151123046875;-0.91636655384152110315199024626053869724273681640625;-1.3820197771531963493174544055364094674587249755859375;-0.57267864066817819601595829226425848901271820068359375;1.5022433235315377775265233140089549124240875244140625;0.923805836263870361335648340173065662384033203125]
      mask Display: e = 0.06;c1 = [120 150 230]/255;c2 = ([120 150 230]+0)/383;c3 = ([120 150 230]+128)/383;patch([0 1 1 0],[0 0 1 1],c1);patch([0 1 1 1-e 1-e 0+e],[0 0 1 1-e 0+e 0+e],c2);patch([0 0 1 1-e 0+e 0+e],[0 1 1 1-e 1-e 0+e],c3);plot([0 1 1 0 0],[0 0 1 1 0]);disp('weights');
  "IW{2,1}(582,:)'" : Constant  Value=[-0.97587104860400442074563898131600581109523773193359375;-1.6677548525125323042317404542700387537479400634765625;-0.481625163390215271785876893773092888295650482177734375;0.50985104988977891782298001999151892960071563720703125;-1.693589027418287429327392601408064365386962890625;-0.559512341061640494643825149978511035442352294921875;-1.73735844261201055616083976929076015949249267578125;0.76157420951346377346879990000161342322826385498046875]
      mask Display: e = 0.06;c1 = [120 150 230]/255;c2 = ([120 150 230]+0)/383;c3 = ([120 150 230]+128)/383;patch([0 1 1 0],[0 0 1 1],c1);patch([0 1 1 1-e 1-e 0+e],[0 0 1 1-e 0+e 0+e],c2);patch([0 0 1 1-e 0+e 0+e],[0 1 1 1-e 1-e 0+e],c3);plot([0 1 1 0 0],[0 0 1 1 0]);disp('weights');
  "IW{2,1}(583,:)'" : Constant  Value=[0.182382386697061971148059456027112901210784912109375;-1.44316655298723528488835654570721089839935302734375;-0.481706885832457631924086172148236073553562164306640625;1.5444552448286674728450407201307825744152069091796875;-1.231389565646216599503759425715543329715728759765625;-0.2617167289911523919698765894281677901744842529296875;1.6878955206222332474652603195863775908946990966796875;-1.5001379074035401384179522210615687072277069091796875]
      mask Display: e = 0.06;c1 = [120 150 230]/255;c2 = ([120 150 230]+0)/383;c3 = ([120 150 230]+128)/383;patch([0 1 1 0],[0 0 1 1],c1);patch([0 1 1 1-e 1-e 0+e],[0 0 1 1-e 0+e 0+e],c2);patch([0 0 1 1-e 0+e 0+e],[0 1 1 1-e 1-e 0+e],c3);plot([0 1 1 0 0],[0 0 1 1 0]);disp('weights');
  "IW{2,1}(584,:)'" : Constant  Value=[1.0236053268348559441847100970335304737091064453125;-2.142793453662150238159256332437507808208465576171875;-0.1902181357051813404002160723393899388611316680908203125;-1.59272752436353126626045195735059678554534912109375;0.87624476074240498224554585249279625713825225830078125;-1.0950430264665962365455698090954683721065521240234375;-0.65006824336162527533389265954610891640186309814453125;0.55099142354084407191550099014420993626117706298828125]
      mask Display: e = 0.06;c1 = [120 150 230]/255;c2 = ([120 150 230]+0)/383;c3 = ([120 150 230]+128)/383;patch([0 1 1 0],[0 0 1 1],c1);patch([0 1 1 1-e 1-e 0+e],[0 0 1 1-e 0+e 0+e],c2);patch([0 0 1 1-e 0+e 0+e],[0 1 1 1-e 1-e 0+e],c3);plot([0 1 1 0 0],[0 0 1 1 0]);disp('weights');
  "IW{2,1}(585,:)'" : Constant  Value=[2.0320933753924617093389315414242446422576904296875;1.6437665296450780783032996623660437762737274169921875;0.812806470795902402670662922901101410388946533203125;1.4956465960466631681669014142244122922420501708984375;-0.95638146773530241517846661736257374286651611328125;-0.005027963694957217517800263095750779029913246631622314453125;0.5459505768224846011804629597463645040988922119140625;-0.37406691828470772787085252275574021041393280029296875]
      mask Display: e = 0.06;c1 = [120 150 230]/255;c2 = ([120 150 230]+0)/383;c3 = ([120 150 230]+128)/383;patch([0 1 1 0],[0 0 1 1],c1);patch([0 1 1 1-e 1-e 0+e],[0 0 1 1-e 0+e 0+e],c2);patch([0 0 1 1-e 0+e 0+e],[0 1 1 1-e 1-e 0+e],c3);plot([0 1 1 0 0],[0 0 1 1 0]);disp('weights');
  "IW{2,1}(586,:)'" : Constant  Value=[0.65092739382151953986266335050459019839763641357421875;0.987225828133180272061508730985224246978759765625;-2.004875456412777534609404028742574155330657958984375;-1.1557756236680500894209444595617242157459259033203125;-0.339149421527736916193163096977514214813709259033203125;-1.2403435713567498854814630249165929853916168212890625;-0.51084435640717540394462048425339162349700927734375;1.5002419401692563827310777924139983952045440673828125]
      mask Display: e = 0.06;c1 = [120 150 230]/255;c2 = ([120 150 230]+0)/383;c3 = ([120 150 230]+128)/383;patch([0 1 1 0],[0 0 1 1],c1);patch([0 1 1 1-e 1-e 0+e],[0 0 1 1-e 0+e 0+e],c2);patch([0 0 1 1-e 0+e 0+e],[0 1 1 1-e 1-e 0+e],c3);plot([0 1 1 0 0],[0 0 1 1 0]);disp('weights');
  "IW{2,1}(587,:)'" : Constant  Value=[1.43820450969185298362162939156405627727508544921875;-1.4016810113738087384405162083567120134830474853515625;0.6143846046343057754057781494338996708393096923828125;-0.82612454159124759645038693633978255093097686767578125;1.5255953200751417586644720358890481293201446533203125;-1.496048787459802298371869255788624286651611328125;0.73179633068911142945722758668125607073307037353515625;-0.94474462440853856914912967113195918500423431396484375]
      mask Display: e = 0.06;c1 = [120 150 230]/255;c2 = ([120 150 230]+0)/383;c3 = ([120 150 230]+128)/383;patch([0 1 1 0],[0 0 1 1],c1);patch([0 1 1 1-e 1-e 0+e],[0 0 1 1-e 0+e 0+e],c2);patch([0 0 1 1-e 0+e 0+e],[0 1 1 1-e 1-e 0+e],c3);plot([0 1 1 0 0],[0 0 1 1 0]);disp('weights');
  "IW{2,1}(588,:)'" : Constant  Value=[-0.09397777380344791986477304135405574925243854522705078125;1.39179462997646385957750680972822010517120361328125;1.1480378085366307328030188728007487952709197998046875;1.3712225921575595943835423895507119596004486083984375;1.1479703559129703638319597303052432835102081298828125;-1.2967491060887663678613535012118518352508544921875;-1.0408617416088954410469114009174518287181854248046875;1.3770403058006761565223996512941084802150726318359375]
      mask Display: e = 0.06;c1 = [120 150 230]/255;c2 = ([120 150 230]+0)/383;c3 = ([120 150 230]+128)/383;patch([0 1 1 0],[0 0 1 1],c1);patch([0 1 1 1-e 1-e 0+e],[0 0 1 1-e 0+e 0+e],c2);patch([0 0 1 1-e 0+e 0+e],[0 1 1 1-e 1-e 0+e],c3);plot([0 1 1 0 0],[0 0 1 1 0]);disp('weights');
  "IW{2,1}(589,:)'" : Constant  Value=[2.01972140642401054577703689574263989925384521484375;-0.35133266461696288640581542495056055486202239990234375;0.96134485545835157704885887142154388129711151123046875;2.3792888026401186607472482137382030487060546875;0.12079478134691283564006170081484015099704265594482421875;0.474077165156534252599129786176490597426891326904296875;-0.33413371838487992970812001658487133681774139404296875;0.0574991573698209190723673600587062537670135498046875]
      mask Display: e = 0.06;c1 = [120 150 230]/255;c2 = ([120 150 230]+0)/383;c3 = ([120 150 230]+128)/383;patch([0 1 1 0],[0 0 1 1],c1);patch([0 1 1 1-e 1-e 0+e],[0 0 1 1-e 0+e 0+e],c2);patch([0 0 1 1-e 0+e 0+e],[0 1 1 1-e 1-e 0+e],c3);plot([0 1 1 0 0],[0 0 1 1 0]);disp('weights');
